simulink model "model_compatible"  (Simulink 7.5)
(part 5 of 5)

  Boundary___Perseus_1_CN_92348290_275000_CN_92343043_275000/RConn2 -- T_92343043_275000_Boundary_Substation/LConn2 -- _CN_92343043_275000_CN_191269219_275000/LConn2
  Boundary___Perseus_1_CN_92348290_275000_CN_92343043_275000/RConn3 -- T_92343043_275000_Boundary_Substation/LConn3 -- _CN_92343043_275000_CN_191269219_275000/LConn3 -- bus101/LConn1
  T_217505021__/LConn1 -- _CN_92348290_275000_CN_217505021_275000/RConn1
  T_217505021__/LConn2 -- _CN_92348290_275000_CN_217505021_275000/RConn2
  _CN_92348290_275000_CN_217505021_275000/RConn3 -- T_217505021__/LConn3 -- bus102/LConn1
  _CN_92343043_275000_CN_191269219_275000/RConn1 -- T_191269219_275000_/LConn1 -- _CN_200757306_275000_CN_191269219_275000/LConn1
  _CN_92343043_275000_CN_191269219_275000/RConn2 -- T_191269219_275000_/LConn2 -- _CN_200757306_275000_CN_191269219_275000/LConn2
  _CN_92343043_275000_CN_191269219_275000/RConn3 -- T_191269219_275000_/LConn3 -- _CN_200757306_275000_CN_191269219_275000/LConn3 -- bus103/LConn1
  T_230551819__/RConn1 -- _CN_230551819_275000_CN_182253896_275000/LConn1
  T_230551819__/RConn2 -- _CN_230551819_275000_CN_182253896_275000/LConn2
  _CN_230551819_275000_CN_182253896_275000/LConn3 -- T_230551819__/RConn3 -- bus104/LConn1
  _CN_230551819_275000_CN_182253896_275000/RConn1 -- T_182253896__/LConn1 -- _CN_182262936_275000_CN_182253896_275000/RConn1
  _CN_230551819_275000_CN_182253896_275000/RConn2 -- T_182253896__/LConn2 -- _CN_182262936_275000_CN_182253896_275000/RConn2
  _CN_230551819_275000_CN_182253896_275000/RConn3 -- T_182253896__/LConn3 -- _CN_182262936_275000_CN_182253896_275000/RConn3 -- bus105/LConn1
  _CN_184191239_275000_CN_107391770_275000/LConn1 -- T_184191239_275000_Illovo_Substation/LConn1 -- _CN_184191239_275000_CN_176259936_275000/LConn1
  _CN_184191239_275000_CN_107391770_275000/LConn2 -- T_184191239_275000_Illovo_Substation/LConn2 -- _CN_184191239_275000_CN_176259936_275000/LConn2
  _CN_184191239_275000_CN_107391770_275000/LConn3 -- T_184191239_275000_Illovo_Substation/LConn3 -- _CN_184191239_275000_CN_176259936_275000/LConn3 -- bus106/LConn1
  _CN_184191239_275000_CN_107391770_275000/RConn1 -- T_107391770_400000;275000_/RConn1 -- _CN_107391770_275000_CN_184187955_275000/LConn1 -- L_107391770/LConn1
  _CN_184191239_275000_CN_107391770_275000/RConn2 -- T_107391770_400000;275000_/RConn2 -- _CN_107391770_275000_CN_184187955_275000/LConn2 -- L_107391770/LConn2
  _CN_184191239_275000_CN_107391770_275000/RConn3 -- T_107391770_400000;275000_/RConn3 -- _CN_107391770_275000_CN_184187955_275000/LConn3 -- L_107391770/LConn3 -- bus107/LConn1
  _CN_184191239_275000_CN_176259936_275000/RConn1 -- T_176259936_275000_Georgedale_Substation/LConn1 -- _CN_184187955_275000_CN_176259936_275000/LConn1 -- _CN_181284056_275000_CN_176259936_275000/LConn1 -- _CN_127585817_275000_CN_176259936_275000/LConn1
  _CN_184191239_275000_CN_176259936_275000/RConn2 -- T_176259936_275000_Georgedale_Substation/LConn2 -- _CN_184187955_275000_CN_176259936_275000/LConn2 -- _CN_181284056_275000_CN_176259936_275000/LConn2 -- _CN_127585817_275000_CN_176259936_275000/LConn2
  _CN_184191239_275000_CN_176259936_275000/RConn3 -- T_176259936_275000_Georgedale_Substation/LConn3 -- _CN_184187955_275000_CN_176259936_275000/LConn3 -- _CN_181284056_275000_CN_176259936_275000/LConn3 -- bus108/LConn1 -- _CN_127585817_275000_CN_176259936_275000/LConn3
  T_184336448__/LConn1 -- _CN_184336448_275000_CN_87404898_275000/RConn1
  T_184336448__/LConn2 -- _CN_184336448_275000_CN_87404898_275000/RConn2
  _CN_184336448_275000_CN_87404898_275000/RConn3 -- T_184336448__/LConn3 -- bus109/LConn1
  T_84274092_380000;132000_/LConn1 -- _CN_84274092_275000_CN_83525879_275000/LConn1
  T_84274092_380000;132000_/LConn2 -- _CN_84274092_275000_CN_83525879_275000/LConn2
  _CN_84274092_275000_CN_83525879_275000/LConn3 -- T_84274092_380000;132000_/LConn3 -- bus110/LConn1
  _CN_84274092_275000_CN_83525879_275000/RConn1 -- T_83525879_400000;275000_Apollo_Substation/RConn1 -- _CN_28088740_275000_CN_83525879_275000/LConn1 -- _CN_83951788_275000_CN_83525879_275000/LConn1 -- _CN_83525876_275000_CN_83525879_275000/LConn1 -- L_83525879/LConn1
  _CN_84274092_275000_CN_83525879_275000/RConn2 -- T_83525879_400000;275000_Apollo_Substation/RConn2 -- _CN_28088740_275000_CN_83525879_275000/LConn2 -- _CN_83951788_275000_CN_83525879_275000/LConn2 -- _CN_83525876_275000_CN_83525879_275000/LConn2 -- L_83525879/LConn2
  _CN_84274092_275000_CN_83525879_275000/RConn3 -- T_83525879_400000;275000_Apollo_Substation/RConn3 -- _CN_28088740_275000_CN_83525879_275000/LConn3 -- _CN_83951788_275000_CN_83525879_275000/LConn3 -- _CN_83525876_275000_CN_83525879_275000/LConn3 -- L_83525879/LConn3 -- bus111/LConn1
  _CN_215459082_275000_CN_149126524_275000/LConn1 -- T_215459082_275000_Rigi_Substation/LConn1 -- _CN_215459082_275000_CN_98231341_275000/LConn1
  _CN_215459082_275000_CN_149126524_275000/LConn2 -- T_215459082_275000_Rigi_Substation/LConn2 -- _CN_215459082_275000_CN_98231341_275000/LConn2
  _CN_215459082_275000_CN_149126524_275000/LConn3 -- T_215459082_275000_Rigi_Substation/LConn3 -- _CN_215459082_275000_CN_98231341_275000/LConn3 -- bus112/LConn1
  _CN_215459082_275000_CN_149126524_275000/RConn1 -- T_149126524_275000_/LConn1 -- _CN_178252032_275000_CN_149126524_275000/LConn1 -- _CN_105811523_275000_CN_149126524_275000/LConn1
  _CN_215459082_275000_CN_149126524_275000/RConn2 -- T_149126524_275000_/LConn2 -- _CN_178252032_275000_CN_149126524_275000/LConn2 -- _CN_105811523_275000_CN_149126524_275000/LConn2
  _CN_215459082_275000_CN_149126524_275000/RConn3 -- T_149126524_275000_/LConn3 -- _CN_178252032_275000_CN_149126524_275000/LConn3 -- bus113/LConn1 -- _CN_105811523_275000_CN_149126524_275000/LConn3
  _CN_215459082_275000_CN_98231341_275000/RConn1 -- T_98231341_275000_/LConn1 -- _CN_98231341_275000_CN_214437948_275000/LConn1 -- _CN_98231341_275000_CN_136695854_275000/LConn1 -- _CN_98231341_275000_CN_105811523_275000/LConn1 -- _CN_98231341_275000_CN_81817181_275000/LConn1 -- _CN_98231341_275000_CN_189739076_275000/LConn1
  _CN_215459082_275000_CN_98231341_275000/RConn2 -- T_98231341_275000_/LConn2 -- _CN_98231341_275000_CN_214437948_275000/LConn2 -- _CN_98231341_275000_CN_136695854_275000/LConn2 -- _CN_98231341_275000_CN_105811523_275000/LConn2 -- _CN_98231341_275000_CN_81817181_275000/LConn2 -- _CN_98231341_275000_CN_189739076_275000/LConn2
  _CN_215459082_275000_CN_98231341_275000/RConn3 -- T_98231341_275000_/LConn3 -- _CN_98231341_275000_CN_214437948_275000/LConn3 -- _CN_98231341_275000_CN_136695854_275000/LConn3 -- _CN_98231341_275000_CN_105811523_275000/LConn3 -- _CN_98231341_275000_CN_81817181_275000/LConn3 -- _CN_98231341_275000_CN_189739076_275000/LConn3 -- bus114/LConn1
  _CN_183907671_275000_CN_181284049_275000/LConn1 -- T_183907671_275000;132000_Avon_Substation/LConn1 -- _CN_183907671_275000_CN_183907662_275000/LConn1
  _CN_183907671_275000_CN_181284049_275000/LConn2 -- T_183907671_275000;132000_Avon_Substation/LConn2 -- _CN_183907671_275000_CN_183907662_275000/LConn2
  _CN_183907671_275000_CN_181284049_275000/LConn3 -- T_183907671_275000;132000_Avon_Substation/LConn3 -- _CN_183907671_275000_CN_183907662_275000/LConn3 -- bus115/LConn1
  T_181284049__/RConn1 -- _CN_183907671_275000_CN_181284049_275000/RConn1
  T_181284049__/RConn2 -- _CN_183907671_275000_CN_181284049_275000/RConn2
  _CN_183907671_275000_CN_181284049_275000/RConn3 -- T_181284049__/RConn3 -- bus116/LConn1
  T_183907662_275000;132000_Ottawa_Substation/LConn1 -- _CN_183907671_275000_CN_183907662_275000/RConn1
  T_183907662_275000;132000_Ottawa_Substation/LConn2 -- _CN_183907671_275000_CN_183907662_275000/RConn2
  _CN_183907671_275000_CN_183907662_275000/RConn3 -- T_183907662_275000;132000_Ottawa_Substation/LConn3 -- bus117/LConn1
  T_184602696__/LConn1 -- _CN_184602696_275000_CN_184552955_275000/LConn1
  T_184602696__/LConn2 -- _CN_184602696_275000_CN_184552955_275000/LConn2
  _CN_184602696_275000_CN_184552955_275000/LConn3 -- T_184602696__/LConn3 -- bus118/LConn1
  _CN_184602696_275000_CN_184552955_275000/RConn1 -- T_184552955__/RConn1 -- _CN_258020275_275000_CN_184552955_275000/LConn1 -- _CN_184552955_275000_CN_208749745_275000/LConn1 -- L_184552955/LConn1
  _CN_184602696_275000_CN_184552955_275000/RConn2 -- T_184552955__/RConn2 -- _CN_258020275_275000_CN_184552955_275000/LConn2 -- _CN_184552955_275000_CN_208749745_275000/LConn2 -- L_184552955/LConn2
  _CN_184602696_275000_CN_184552955_275000/RConn3 -- T_184552955__/RConn3 -- _CN_258020275_275000_CN_184552955_275000/LConn3 -- _CN_184552955_275000_CN_208749745_275000/LConn3 -- L_184552955/LConn3 -- bus119/LConn1
  _CN_75136015_275000_CN_32509808_275000/LConn1 -- T_75136015_400000;275000_Minerva_Substation/RConn1 -- _CN_75136015_275000_CN_187432497_275000/LConn1 -- L_75136015/LConn1 -- _CN_75136015_275000_CN_178950118_275000/LConn1 -- _CN_75136015_275000_CN_84197405_275000/LConn1
  _CN_75136015_275000_CN_32509808_275000/LConn2 -- T_75136015_400000;275000_Minerva_Substation/RConn2 -- _CN_75136015_275000_CN_187432497_275000/LConn2 -- L_75136015/LConn2 -- _CN_75136015_275000_CN_178950118_275000/LConn2 -- _CN_75136015_275000_CN_84197405_275000/LConn2
  _CN_75136015_275000_CN_32509808_275000/LConn3 -- T_75136015_400000;275000_Minerva_Substation/RConn3 -- _CN_75136015_275000_CN_187432497_275000/LConn3 -- L_75136015/LConn3 -- bus120/LConn1 -- _CN_75136015_275000_CN_178950118_275000/LConn3 -- _CN_75136015_275000_CN_84197405_275000/LConn3
  _CN_75136015_275000_CN_32509808_275000/RConn1 -- T_32509808__Lepini_Substation/LConn1 -- _CN_178950118_275000_CN_32509808_275000/LConn1
  _CN_75136015_275000_CN_32509808_275000/RConn2 -- T_32509808__Lepini_Substation/LConn2 -- _CN_178950118_275000_CN_32509808_275000/LConn2
  _CN_75136015_275000_CN_32509808_275000/RConn3 -- T_32509808__Lepini_Substation/LConn3 -- _CN_178950118_275000_CN_32509808_275000/LConn3 -- bus121/LConn1
  _CN_75136015_275000_CN_178950118_275000/RConn1 -- T_178950118_275000_Craighall_Substation/LConn1 -- _CN_178950118_275000_CN_32509808_275000/RConn1
  _CN_75136015_275000_CN_178950118_275000/RConn2 -- T_178950118_275000_Craighall_Substation/LConn2 -- _CN_178950118_275000_CN_32509808_275000/RConn2
  _CN_75136015_275000_CN_178950118_275000/RConn3 -- T_178950118_275000_Craighall_Substation/LConn3 -- _CN_178950118_275000_CN_32509808_275000/RConn3 -- bus122/LConn1
  T_84197405_380000;132000_/LConn1 -- _CN_75136015_275000_CN_84197405_275000/RConn1
  T_84197405_380000;132000_/LConn2 -- _CN_75136015_275000_CN_84197405_275000/RConn2
  _CN_75136015_275000_CN_84197405_275000/RConn3 -- T_84197405_380000;132000_/LConn3 -- bus123/LConn1
  T_187432497__/LConn1 -- _CN_75136015_275000_CN_187432497_275000/RConn1
  T_187432497__/LConn2 -- _CN_75136015_275000_CN_187432497_275000/RConn2
  _CN_75136015_275000_CN_187432497_275000/RConn3 -- T_187432497__/LConn3 -- bus124/LConn1
  _CN_156418705_275000_CN_136019706_275000/RConn1 -- T_136019706__/LConn1 -- _CN_135726365_275000_CN_136019706_275000/LConn1
  _CN_156418705_275000_CN_136019706_275000/RConn2 -- T_136019706__/LConn2 -- _CN_135726365_275000_CN_136019706_275000/LConn2
  _CN_156418705_275000_CN_136019706_275000/RConn3 -- T_136019706__/LConn3 -- _CN_135726365_275000_CN_136019706_275000/LConn3 -- bus125/LConn1
  T_247956792__/LConn1 -- _CN_247956792_275000_CN_183764510_275000/LConn1
  T_247956792__/LConn2 -- _CN_247956792_275000_CN_183764510_275000/LConn2
  _CN_247956792_275000_CN_183764510_275000/LConn3 -- T_247956792__/LConn3 -- bus126/LConn1
  T_183764510__/LConn1 -- _CN_247956792_275000_CN_183764510_275000/RConn1
  T_183764510__/LConn2 -- _CN_247956792_275000_CN_183764510_275000/RConn2
  _CN_247956792_275000_CN_183764510_275000/RConn3 -- T_183764510__/LConn3 -- bus127/LConn1
  _CN_178987907_275000_CN_418832508_275000/RConn1 -- G_418832508_Arnot_Power_Station/RConn1 -- _CN_156418705_400000_CN_418832508_275000/LConn1 -- _CN_170672051_400000_CN_418832508_275000/LConn1 -- _CN_209976655_400000_CN_418832508_275000/LConn1 -- _CN_220129604_400000_CN_418832508_275000/LConn1
  _CN_178987907_275000_CN_418832508_275000/RConn2 -- G_418832508_Arnot_Power_Station/RConn2 -- _CN_156418705_400000_CN_418832508_275000/LConn2 -- _CN_170672051_400000_CN_418832508_275000/LConn2 -- _CN_209976655_400000_CN_418832508_275000/LConn2 -- _CN_220129604_400000_CN_418832508_275000/LConn2
  _CN_178987907_275000_CN_418832508_275000/RConn3 -- G_418832508_Arnot_Power_Station/RConn3 -- _CN_156418705_400000_CN_418832508_275000/LConn3 -- _CN_170672051_400000_CN_418832508_275000/LConn3 -- _CN_209976655_400000_CN_418832508_275000/LConn3 -- _CN_220129604_400000_CN_418832508_275000/LConn3 -- bus128/LConn1
  T_363326105__/LConn1 -- _CN_363326105_275000_CN_179856840_275000/LConn1
  T_363326105__/LConn2 -- _CN_363326105_275000_CN_179856840_275000/LConn2
  _CN_363326105_275000_CN_179856840_275000/LConn3 -- T_363326105__/LConn3 -- bus129/LConn1
  T_179856840_275000_Komatipoort_Substation/LConn1 -- _CN_363326105_275000_CN_179856840_275000/RConn1
  T_179856840_275000_Komatipoort_Substation/LConn2 -- _CN_363326105_275000_CN_179856840_275000/RConn2
  _CN_363326105_275000_CN_179856840_275000/RConn3 -- T_179856840_275000_Komatipoort_Substation/LConn3 -- bus130/LConn1
  _CN_127585817_275000_CN_176259936_275000/RConn1 -- T_127585817__/RConn1 -- _CN_127585817_275000_CN_148830396_275000/LConn1 -- L_127585817/LConn1
  _CN_127585817_275000_CN_176259936_275000/RConn2 -- T_127585817__/RConn2 -- _CN_127585817_275000_CN_148830396_275000/LConn2 -- L_127585817/LConn2
  _CN_127585817_275000_CN_176259936_275000/RConn3 -- T_127585817__/RConn3 -- _CN_127585817_275000_CN_148830396_275000/LConn3 -- L_127585817/LConn3 -- bus131/LConn1
  _CN_127585817_275000_CN_148830396_275000/RConn1 -- T_148830396__/LConn1 -- _CN_104071861_275000_CN_148830396_275000/LConn1
  _CN_127585817_275000_CN_148830396_275000/RConn2 -- T_148830396__/LConn2 -- _CN_104071861_275000_CN_148830396_275000/LConn2
  _CN_127585817_275000_CN_148830396_275000/RConn3 -- T_148830396__/LConn3 -- _CN_104071861_275000_CN_148830396_275000/LConn3 -- bus132/LConn1
  _CN_84391364_275000_CN_136695854_275000/LConn1 -- T_84391364_275000_Nevis_Substation/LConn1 -- _CN_84391364_275000_CN_418842091_275000/LConn1 -- _CN_84391364_275000_CN_136695855_275000/LConn1
  _CN_84391364_275000_CN_136695854_275000/LConn2 -- T_84391364_275000_Nevis_Substation/LConn2 -- _CN_84391364_275000_CN_418842091_275000/LConn2 -- _CN_84391364_275000_CN_136695855_275000/LConn2
  _CN_84391364_275000_CN_136695854_275000/LConn3 -- T_84391364_275000_Nevis_Substation/LConn3 -- _CN_84391364_275000_CN_418842091_275000/LConn3 -- bus133/LConn1 -- _CN_84391364_275000_CN_136695855_275000/LConn3
  _CN_84391364_275000_CN_136695854_275000/RConn1 -- T_136695854__/LConn1 -- _CN_98231341_275000_CN_136695854_275000/RConn1
  _CN_84391364_275000_CN_136695854_275000/RConn2 -- T_136695854__/LConn2 -- _CN_98231341_275000_CN_136695854_275000/RConn2
  _CN_84391364_275000_CN_136695854_275000/RConn3 -- T_136695854__/LConn3 -- _CN_98231341_275000_CN_136695854_275000/RConn3 -- bus134/LConn1
  T_136695855__/LConn1 -- _CN_84391364_275000_CN_136695855_275000/RConn1
  T_136695855__/LConn2 -- _CN_84391364_275000_CN_136695855_275000/RConn2
  _CN_84391364_275000_CN_136695855_275000/RConn3 -- T_136695855__/LConn3 -- bus135/LConn1
  _CN_84391364_275000_CN_418842091_275000/RConn1 -- G_418842091_Matla_Power_Station/RConn1 -- _CN_185481654_275000_CN_418842091_275000/LConn1 -- _CN_83950316_275000_CN_418842091_275000/LConn1
  _CN_84391364_275000_CN_418842091_275000/RConn2 -- G_418842091_Matla_Power_Station/RConn2 -- _CN_185481654_275000_CN_418842091_275000/LConn2 -- _CN_83950316_275000_CN_418842091_275000/LConn2
  _CN_84391364_275000_CN_418842091_275000/RConn3 -- G_418842091_Matla_Power_Station/RConn3 -- _CN_185481654_275000_CN_418842091_275000/LConn3 -- _CN_83950316_275000_CN_418842091_275000/LConn3 -- bus136/LConn1
  _CN_107391770_275000_CN_184187955_275000/RConn1 -- T_184187955_275000_Klaarwater_Substation/LConn1 -- _CN_197060002_275000_CN_184187955_275000/LConn1 -- _CN_184187955_275000_CN_176259936_275000/RConn1
  _CN_107391770_275000_CN_184187955_275000/RConn2 -- T_184187955_275000_Klaarwater_Substation/LConn2 -- _CN_197060002_275000_CN_184187955_275000/LConn2 -- _CN_184187955_275000_CN_176259936_275000/RConn2
  _CN_107391770_275000_CN_184187955_275000/RConn3 -- T_184187955_275000_Klaarwater_Substation/LConn3 -- _CN_197060002_275000_CN_184187955_275000/LConn3 -- _CN_184187955_275000_CN_176259936_275000/RConn3 -- bus137/LConn1
  T_178240540__/LConn1 -- _CN_178240540_275000_CN_83188568_275000/LConn1
  T_178240540__/LConn2 -- _CN_178240540_275000_CN_83188568_275000/LConn2
  _CN_178240540_275000_CN_83188568_275000/LConn3 -- T_178240540__/LConn3 -- bus138/LConn1
  _CN_178240540_275000_CN_83188568_275000/RConn1 -- T_83188568_275000;132000_Taunus_Substation/LConn1 -- _CN_178240552_275000_CN_83188568_275000/LConn1 -- _CN_83888980_275000_CN_83188568_275000/LConn1 -- _CN_82014905_275000_CN_83188568_275000/LConn1
  _CN_178240540_275000_CN_83188568_275000/RConn2 -- T_83188568_275000;132000_Taunus_Substation/LConn2 -- _CN_178240552_275000_CN_83188568_275000/LConn2 -- _CN_83888980_275000_CN_83188568_275000/LConn2 -- _CN_82014905_275000_CN_83188568_275000/LConn2
  _CN_178240540_275000_CN_83188568_275000/RConn3 -- T_83188568_275000;132000_Taunus_Substation/LConn3 -- _CN_178240552_275000_CN_83188568_275000/LConn3 -- _CN_83888980_275000_CN_83188568_275000/LConn3 -- _CN_82014905_275000_CN_83188568_275000/LConn3 -- bus139/LConn1
  T_100421919__/LConn1 -- _CN_100421919_275000_CN_200757306_275000/LConn1
  T_100421919__/LConn2 -- _CN_100421919_275000_CN_200757306_275000/LConn2
  _CN_100421919_275000_CN_200757306_275000/LConn3 -- T_100421919__/LConn3 -- bus140/LConn1
  _CN_100421919_275000_CN_200757306_275000/RConn1 -- T_200757306__/LConn1 -- _CN_200757306_275000_CN_191269219_275000/RConn1
  _CN_100421919_275000_CN_200757306_275000/RConn2 -- T_200757306__/LConn2 -- _CN_200757306_275000_CN_191269219_275000/RConn2
  _CN_100421919_275000_CN_200757306_275000/RConn3 -- T_200757306__/LConn3 -- _CN_200757306_275000_CN_191269219_275000/RConn3 -- bus141/LConn1
  _CN_131625968_275000_CN_120941257_275000/LConn1 -- T_131625968_132000_Nseleni_Substation/RConn1 -- L_131625968/LConn1
  _CN_131625968_275000_CN_120941257_275000/LConn2 -- T_131625968_132000_Nseleni_Substation/RConn2 -- L_131625968/LConn2
  _CN_131625968_275000_CN_120941257_275000/LConn3 -- T_131625968_132000_Nseleni_Substation/RConn3 -- L_131625968/LConn3 -- bus142/LConn1
  T_120941257_275000;132000_Impala_Substation/LConn1 -- _CN_131625968_275000_CN_120941257_275000/RConn1
  T_120941257_275000;132000_Impala_Substation/LConn2 -- _CN_131625968_275000_CN_120941257_275000/RConn2
  _CN_131625968_275000_CN_120941257_275000/RConn3 -- T_120941257_275000;132000_Impala_Substation/LConn3 -- bus143/LConn1
  T_197060002__/LConn1 -- _CN_197060002_275000_CN_184187955_275000/RConn1
  T_197060002__/LConn2 -- _CN_197060002_275000_CN_184187955_275000/RConn2
  _CN_197060002_275000_CN_184187955_275000/RConn3 -- T_197060002__/LConn3 -- bus144/LConn1
  _CN_220129604_275000_CN_101150274_275000/LConn1 -- T_220129604_400000_Arnot_Power_Station/RConn1 -- _CN_220129604_275000_CN_138280477_275000/LConn1 -- L_220129604/LConn1
  _CN_220129604_275000_CN_101150274_275000/LConn2 -- T_220129604_400000_Arnot_Power_Station/RConn2 -- _CN_220129604_275000_CN_138280477_275000/LConn2 -- L_220129604/LConn2
  _CN_220129604_275000_CN_101150274_275000/LConn3 -- T_220129604_400000_Arnot_Power_Station/RConn3 -- _CN_220129604_275000_CN_138280477_275000/LConn3 -- L_220129604/LConn3 -- bus145/LConn1
  _CN_220129604_275000_CN_101150274_275000/RConn1 -- T_101150274__/LConn1 -- _CN_93158442_275000_CN_101150274_275000/LConn1
  _CN_220129604_275000_CN_101150274_275000/RConn2 -- T_101150274__/LConn2 -- _CN_93158442_275000_CN_101150274_275000/LConn2
  _CN_220129604_275000_CN_101150274_275000/RConn3 -- T_101150274__/LConn3 -- _CN_93158442_275000_CN_101150274_275000/LConn3 -- bus146/LConn1
  T_138280477__/LConn1 -- _CN_220129604_275000_CN_138280477_275000/RConn1
  T_138280477__/LConn2 -- _CN_220129604_275000_CN_138280477_275000/RConn2
  _CN_220129604_275000_CN_138280477_275000/RConn3 -- T_138280477__/LConn3 -- bus147/LConn1
  _CN_28088740_275000_CN_83525879_275000/RConn1 -- T_28088740_275000_Croydon_Substation/LConn1 -- _CN_28088740_275000_CN_42209860_275000/LConn1
  _CN_28088740_275000_CN_83525879_275000/RConn2 -- T_28088740_275000_Croydon_Substation/LConn2 -- _CN_28088740_275000_CN_42209860_275000/LConn2
  _CN_28088740_275000_CN_83525879_275000/RConn3 -- T_28088740_275000_Croydon_Substation/LConn3 -- _CN_28088740_275000_CN_42209860_275000/LConn3 -- bus148/LConn1
  _CN_28088740_275000_CN_42209860_275000/RConn1 -- T_42209860_275000_Jupiter_Substation/LConn1 -- _CN_42209860_275000_CN_42209493_275000/LConn1 -- _CN_42209860_275000_CN_178944143_275000/LConn1
  _CN_28088740_275000_CN_42209860_275000/RConn2 -- T_42209860_275000_Jupiter_Substation/LConn2 -- _CN_42209860_275000_CN_42209493_275000/LConn2 -- _CN_42209860_275000_CN_178944143_275000/LConn2
  _CN_28088740_275000_CN_42209860_275000/RConn3 -- T_42209860_275000_Jupiter_Substation/LConn3 -- _CN_42209860_275000_CN_42209493_275000/LConn3 -- _CN_42209860_275000_CN_178944143_275000/LConn3 -- bus149/LConn1
  _CN_178240552_275000_CN_105811523_275000/LConn1 -- T_178240552__/LConn1 -- _CN_178240552_275000_CN_83945972_275000/LConn1 -- _CN_178240552_275000_CN_83188568_275000/RConn1
  _CN_178240552_275000_CN_105811523_275000/LConn2 -- T_178240552__/LConn2 -- _CN_178240552_275000_CN_83945972_275000/LConn2 -- _CN_178240552_275000_CN_83188568_275000/RConn2
  _CN_178240552_275000_CN_105811523_275000/LConn3 -- T_178240552__/LConn3 -- _CN_178240552_275000_CN_83945972_275000/LConn3 -- _CN_178240552_275000_CN_83188568_275000/RConn3 -- bus150/LConn1
  _CN_178240552_275000_CN_105811523_275000/RConn1 -- T_105811523_400000;275000_Glockner_Substation/RConn1 -- _CN_98231341_275000_CN_105811523_275000/RConn1 -- _CN_105811509_275000_CN_105811523_275000/LConn1 -- _CN_105811523_275000_CN_178248302_275000/LConn1 -- _CN_105811523_275000_CN_149126524_275000/RConn1 -- L_105811523/LConn1
  _CN_178240552_275000_CN_105811523_275000/RConn2 -- T_105811523_400000;275000_Glockner_Substation/RConn2 -- _CN_98231341_275000_CN_105811523_275000/RConn2 -- _CN_105811509_275000_CN_105811523_275000/LConn2 -- _CN_105811523_275000_CN_178248302_275000/LConn2 -- _CN_105811523_275000_CN_149126524_275000/RConn2 -- L_105811523/LConn2
  _CN_178240552_275000_CN_105811523_275000/RConn3 -- T_105811523_400000;275000_Glockner_Substation/RConn3 -- _CN_98231341_275000_CN_105811523_275000/RConn3 -- _CN_105811509_275000_CN_105811523_275000/LConn3 -- _CN_105811523_275000_CN_178248302_275000/LConn3 -- _CN_105811523_275000_CN_149126524_275000/RConn3 -- L_105811523/LConn3 -- bus151/LConn1
  _CN_178240552_275000_CN_83945972_275000/RConn1 -- T_83945972__/LConn1 -- _CN_83888980_275000_CN_83945972_275000/LConn1
  _CN_178240552_275000_CN_83945972_275000/RConn2 -- T_83945972__/LConn2 -- _CN_83888980_275000_CN_83945972_275000/LConn2
  _CN_178240552_275000_CN_83945972_275000/RConn3 -- T_83945972__/LConn3 -- _CN_83888980_275000_CN_83945972_275000/LConn3 -- bus152/LConn1
  T_93158442_275000_Marathon_Substation/LConn1 -- _CN_93158442_275000_CN_101150274_275000/RConn1
  T_93158442_275000_Marathon_Substation/LConn2 -- _CN_93158442_275000_CN_101150274_275000/RConn2
  _CN_93158442_275000_CN_101150274_275000/RConn3 -- T_93158442_275000_Marathon_Substation/LConn3 -- bus153/LConn1
  _CN_83951788_275000_CN_83525879_275000/RConn1 -- T_83951788_275000_Esselen_Substation/LConn1 -- _CN_83951788_275000_CN_178983951_275000/LConn1
  _CN_83951788_275000_CN_83525879_275000/RConn2 -- T_83951788_275000_Esselen_Substation/LConn2 -- _CN_83951788_275000_CN_178983951_275000/LConn2
  _CN_83951788_275000_CN_83525879_275000/RConn3 -- T_83951788_275000_Esselen_Substation/LConn3 -- _CN_83951788_275000_CN_178983951_275000/LConn3 -- bus154/LConn1
  _CN_83951788_275000_CN_178983951_275000/RConn1 -- T_178983951__/LConn1 -- _CN_258020275_275000_CN_178983951_275000/LConn1
  _CN_83951788_275000_CN_178983951_275000/RConn2 -- T_178983951__/LConn2 -- _CN_258020275_275000_CN_178983951_275000/LConn2
  _CN_83951788_275000_CN_178983951_275000/RConn3 -- T_178983951__/LConn3 -- _CN_258020275_275000_CN_178983951_275000/LConn3 -- bus155/LConn1
  _CN_98231341_275000_CN_214437948_275000/RConn1 -- T_214437948_275000_Brenner_Substation/LConn1 -- _CN_214437948_275000_CN_81817181_275000/LConn1
  _CN_98231341_275000_CN_214437948_275000/RConn2 -- T_214437948_275000_Brenner_Substation/LConn2 -- _CN_214437948_275000_CN_81817181_275000/LConn2
  _CN_98231341_275000_CN_214437948_275000/RConn3 -- T_214437948_275000_Brenner_Substation/LConn3 -- _CN_214437948_275000_CN_81817181_275000/LConn3 -- bus156/LConn1
  _CN_98231341_275000_CN_81817181_275000/RConn1 -- T_81817181_275000_Eiger_Substation/LConn1 -- _CN_82014905_275000_CN_81817181_275000/LConn1 -- _CN_178944143_275000_CN_81817181_275000/LConn1 -- _CN_214437948_275000_CN_81817181_275000/RConn1 -- _CN_42209493_275000_CN_81817181_275000/LConn1
  _CN_98231341_275000_CN_81817181_275000/RConn2 -- T_81817181_275000_Eiger_Substation/LConn2 -- _CN_82014905_275000_CN_81817181_275000/LConn2 -- _CN_178944143_275000_CN_81817181_275000/LConn2 -- _CN_214437948_275000_CN_81817181_275000/RConn2 -- _CN_42209493_275000_CN_81817181_275000/LConn2
  _CN_98231341_275000_CN_81817181_275000/RConn3 -- T_81817181_275000_Eiger_Substation/LConn3 -- _CN_82014905_275000_CN_81817181_275000/LConn3 -- _CN_178944143_275000_CN_81817181_275000/LConn3 -- bus157/LConn1 -- _CN_214437948_275000_CN_81817181_275000/RConn3 -- _CN_42209493_275000_CN_81817181_275000/LConn3
  _CN_98231341_275000_CN_189739076_275000/RConn1 -- T_189739076_275000_Makalu_Substation/LConn1 -- _CN_189739076_275000_CN_178252032_275000/LConn1
  _CN_98231341_275000_CN_189739076_275000/RConn2 -- T_189739076_275000_Makalu_Substation/LConn2 -- _CN_189739076_275000_CN_178252032_275000/LConn2
  _CN_98231341_275000_CN_189739076_275000/RConn3 -- T_189739076_275000_Makalu_Substation/LConn3 -- _CN_189739076_275000_CN_178252032_275000/LConn3 -- bus158/LConn1
  T_135726365__/LConn1 -- _CN_135726365_275000_CN_136019706_275000/RConn1
  T_135726365__/LConn2 -- _CN_135726365_275000_CN_136019706_275000/RConn2
  _CN_135726365_275000_CN_136019706_275000/RConn3 -- T_135726365__/LConn3 -- bus159/LConn1
  T_104071861__/LConn1 -- _CN_104071861_275000_CN_148830396_275000/RConn1
  T_104071861__/LConn2 -- _CN_104071861_275000_CN_148830396_275000/RConn2
  _CN_104071861_275000_CN_148830396_275000/RConn3 -- T_104071861__/LConn3 -- bus160/LConn1
  _CN_185481654_275000_CN_185341298_275000/LConn1 -- T_185481654__/LConn1 -- _CN_185481654_275000_CN_209979772_275000/LConn1 -- _CN_185481654_275000_CN_418842091_275000/RConn1
  _CN_185481654_275000_CN_185341298_275000/LConn2 -- T_185481654__/LConn2 -- _CN_185481654_275000_CN_209979772_275000/LConn2 -- _CN_185481654_275000_CN_418842091_275000/RConn2
  _CN_185481654_275000_CN_185341298_275000/LConn3 -- T_185481654__/LConn3 -- _CN_185481654_275000_CN_209979772_275000/LConn3 -- _CN_185481654_275000_CN_418842091_275000/RConn3 -- bus161/LConn1
  G_185341298_/RConn1 -- _CN_185481654_275000_CN_185341298_275000/RConn1
  G_185341298_/RConn2 -- _CN_185481654_275000_CN_185341298_275000/RConn2
  _CN_185481654_275000_CN_185341298_275000/RConn3 -- G_185341298_/RConn3 -- bus162/LConn1
  T_209979772__/LConn1 -- _CN_185481654_275000_CN_209979772_275000/RConn1
  T_209979772__/LConn2 -- _CN_185481654_275000_CN_209979772_275000/RConn2
  _CN_185481654_275000_CN_209979772_275000/RConn3 -- T_209979772__/LConn3 -- bus163/LConn1
  T_181284056_275000_/LConn1 -- _CN_181284056_275000_CN_176259936_275000/RConn1
  T_181284056_275000_/LConn2 -- _CN_181284056_275000_CN_176259936_275000/RConn2
  _CN_181284056_275000_CN_176259936_275000/RConn3 -- T_181284056_275000_/LConn3 -- bus164/LConn1
  T_83525876__/LConn1 -- _CN_83525876_275000_CN_83525879_275000/RConn1
  T_83525876__/LConn2 -- _CN_83525876_275000_CN_83525879_275000/RConn2
  _CN_83525876_275000_CN_83525879_275000/RConn3 -- T_83525876__/LConn3 -- bus165/LConn1
  T_105811509_275000_Verdun_Substation/LConn1 -- _CN_105811509_275000_CN_105811523_275000/RConn1
  T_105811509_275000_Verdun_Substation/LConn2 -- _CN_105811509_275000_CN_105811523_275000/RConn2
  _CN_105811509_275000_CN_105811523_275000/RConn3 -- T_105811509_275000_Verdun_Substation/LConn3 -- bus166/LConn1
  T_178248302_275000_Kookfontein_Substation/LConn1 -- _CN_105811523_275000_CN_178248302_275000/RConn1
  T_178248302_275000_Kookfontein_Substation/LConn2 -- _CN_105811523_275000_CN_178248302_275000/RConn2
  _CN_105811523_275000_CN_178248302_275000/RConn3 -- T_178248302_275000_Kookfontein_Substation/LConn3 -- bus167/LConn1
  _CN_42209860_275000_CN_42209493_275000/RConn1 -- T_42209493_275000;132000_Prospec_Substation/LConn1 -- _CN_42209493_275000_CN_81817181_275000/RConn1
  _CN_42209860_275000_CN_42209493_275000/RConn2 -- T_42209493_275000;132000_Prospec_Substation/LConn2 -- _CN_42209493_275000_CN_81817181_275000/RConn2
  _CN_42209860_275000_CN_42209493_275000/RConn3 -- T_42209493_275000;132000_Prospec_Substation/LConn3 -- _CN_42209493_275000_CN_81817181_275000/RConn3 -- bus168/LConn1
  _CN_42209860_275000_CN_178944143_275000/RConn1 -- T_178944143_275000_Fordsburg_Substation/LConn1 -- _CN_178944143_275000_CN_81817181_275000/RConn1
  _CN_42209860_275000_CN_178944143_275000/RConn2 -- T_178944143_275000_Fordsburg_Substation/LConn2 -- _CN_178944143_275000_CN_81817181_275000/RConn2
  _CN_42209860_275000_CN_178944143_275000/RConn3 -- T_178944143_275000_Fordsburg_Substation/LConn3 -- _CN_178944143_275000_CN_81817181_275000/RConn3 -- bus169/LConn1
  _CN_189739076_275000_CN_178252032_275000/RConn1 -- T_178252032_275000_Scafell_Substation/LConn1 -- _CN_178252032_275000_CN_149126524_275000/RConn1
  _CN_189739076_275000_CN_178252032_275000/RConn2 -- T_178252032_275000_Scafell_Substation/LConn2 -- _CN_178252032_275000_CN_149126524_275000/RConn2
  _CN_189739076_275000_CN_178252032_275000/RConn3 -- T_178252032_275000_Scafell_Substation/LConn3 -- _CN_178252032_275000_CN_149126524_275000/RConn3 -- bus170/LConn1
  _CN_83888980_275000_CN_83188568_275000/RConn1 -- T_83888980__/LConn1 -- _CN_83888980_275000_CN_83945972_275000/RConn1
  _CN_83888980_275000_CN_83188568_275000/RConn2 -- T_83888980__/LConn2 -- _CN_83888980_275000_CN_83945972_275000/RConn2
  _CN_83888980_275000_CN_83188568_275000/RConn3 -- T_83888980__/LConn3 -- _CN_83888980_275000_CN_83945972_275000/RConn3 -- bus171/LConn1
  _CN_258020275_275000_CN_178983951_275000/RConn1 -- T_258020275__/LConn1 -- _CN_258020275_275000_CN_184552955_275000/RConn1
  _CN_258020275_275000_CN_178983951_275000/RConn2 -- T_258020275__/LConn2 -- _CN_258020275_275000_CN_184552955_275000/RConn2
  _CN_258020275_275000_CN_178983951_275000/RConn3 -- T_258020275__/LConn3 -- _CN_258020275_275000_CN_184552955_275000/RConn3 -- bus172/LConn1
  _CN_82014905_275000_CN_81817181_275000/RConn1 -- T_82014905_275000_Etna_Substation/LConn1 -- _CN_82014905_275000_CN_83188568_275000/RConn1
  _CN_82014905_275000_CN_81817181_275000/RConn2 -- T_82014905_275000_Etna_Substation/LConn2 -- _CN_82014905_275000_CN_83188568_275000/RConn2
  _CN_82014905_275000_CN_81817181_275000/RConn3 -- T_82014905_275000_Etna_Substation/LConn3 -- _CN_82014905_275000_CN_83188568_275000/RConn3 -- bus173/LConn1
  T_208749745__/LConn1 -- _CN_184552955_275000_CN_208749745_275000/RConn1
  T_208749745__/LConn2 -- _CN_184552955_275000_CN_208749745_275000/RConn2
  _CN_184552955_275000_CN_208749745_275000/RConn3 -- T_208749745__/LConn3 -- bus174/LConn1
  T_83950316_275000_Benburg_Substation/LConn1 -- _CN_83950316_275000_CN_418842091_275000/RConn1
  T_83950316_275000_Benburg_Substation/LConn2 -- _CN_83950316_275000_CN_418842091_275000/RConn2
  _CN_83950316_275000_CN_418842091_275000/RConn3 -- T_83950316_275000_Benburg_Substation/LConn3 -- bus175/LConn1
  _CN_176940672_400000_CN_230551819_400000/LConn1 -- T_176940672__/LConn1 -- _CN_176940672_400000_CN_184581460_400000/LConn1
  _CN_176940672_400000_CN_230551819_400000/LConn2 -- T_176940672__/LConn2 -- _CN_176940672_400000_CN_184581460_400000/LConn2
  _CN_176940672_400000_CN_230551819_400000/LConn3 -- T_176940672__/LConn3 -- _CN_176940672_400000_CN_184581460_400000/LConn3 -- bus176/LConn1
  _CN_176940672_400000_CN_230551819_400000/RConn1 -- T_230551819__/LConn1 -- _CN_230551819_400000_CN_182408147_400000/LConn1
  _CN_176940672_400000_CN_230551819_400000/RConn2 -- T_230551819__/LConn2 -- _CN_230551819_400000_CN_182408147_400000/LConn2
  _CN_176940672_400000_CN_230551819_400000/RConn3 -- T_230551819__/LConn3 -- _CN_230551819_400000_CN_182408147_400000/LConn3 -- bus177/LConn1
  _CN_176940672_400000_CN_184581460_400000/RConn1 -- T_184581460__/LConn1 -- _CN_184581460_400000_CN_83525879_400000/LConn1
  _CN_176940672_400000_CN_184581460_400000/RConn2 -- T_184581460__/LConn2 -- _CN_184581460_400000_CN_83525879_400000/LConn2
  _CN_176940672_400000_CN_184581460_400000/RConn3 -- T_184581460__/LConn3 -- _CN_184581460_400000_CN_83525879_400000/LConn3 -- bus178/LConn1
  _CN_185497473_400000_CN_83525879_400000/LConn1 -- T_185497473__/LConn1 -- _CN_185497473_400000_CN_185171511_400000/LConn1 -- _CN_185497473_400000_CN_178968761_400000/LConn1 -- _CN_185497473_400000_CN_75136015_400000/LConn1
  _CN_185497473_400000_CN_83525879_400000/LConn2 -- T_185497473__/LConn2 -- _CN_185497473_400000_CN_185171511_400000/LConn2 -- _CN_185497473_400000_CN_178968761_400000/LConn2 -- _CN_185497473_400000_CN_75136015_400000/LConn2
  _CN_185497473_400000_CN_83525879_400000/LConn3 -- T_185497473__/LConn3 -- _CN_185497473_400000_CN_185171511_400000/LConn3 -- _CN_185497473_400000_CN_178968761_400000/LConn3 -- _CN_185497473_400000_CN_75136015_400000/LConn3 -- bus179/LConn1
  _CN_185497473_400000_CN_83525879_400000/RConn1 -- T_83525879_400000;275000_Apollo_Substation/LConn1 -- _CN_75136015_400000_CN_83525879_400000/LConn1 -- _CN_170672051_400000_CN_83525879_400000/LConn1 -- _CN_185171518_400000_CN_83525879_400000/LConn1 -- _CN_184581460_400000_CN_83525879_400000/RConn1
  _CN_185497473_400000_CN_83525879_400000/RConn2 -- T_83525879_400000;275000_Apollo_Substation/LConn2 -- _CN_75136015_400000_CN_83525879_400000/LConn2 -- _CN_170672051_400000_CN_83525879_400000/LConn2 -- _CN_185171518_400000_CN_83525879_400000/LConn2 -- _CN_184581460_400000_CN_83525879_400000/RConn2
  _CN_185497473_400000_CN_83525879_400000/RConn3 -- T_83525879_400000;275000_Apollo_Substation/LConn3 -- _CN_75136015_400000_CN_83525879_400000/LConn3 -- bus180/LConn1 -- _CN_170672051_400000_CN_83525879_400000/LConn3 -- _CN_185171518_400000_CN_83525879_400000/LConn3 -- _CN_184581460_400000_CN_83525879_400000/RConn3
  _CN_185497473_400000_CN_185171511_400000/RConn1 -- G_185171511_Duvha_Power_Station/RConn1 -- _CN_184560833_400000_CN_185171511_400000/LConn1 -- _CN_238322344_400000_CN_185171511_400000/LConn1 -- _CN_170672051_400000_CN_185171511_400000/LConn1 -- _CN_65600948_400000_CN_185171511_400000/LConn1 -- _CN_185171518_400000_CN_185171511_400000/LConn1
  _CN_185497473_400000_CN_185171511_400000/RConn2 -- G_185171511_Duvha_Power_Station/RConn2 -- _CN_184560833_400000_CN_185171511_400000/LConn2 -- _CN_238322344_400000_CN_185171511_400000/LConn2 -- _CN_170672051_400000_CN_185171511_400000/LConn2 -- _CN_65600948_400000_CN_185171511_400000/LConn2 -- _CN_185171518_400000_CN_185171511_400000/LConn2
  _CN_185497473_400000_CN_185171511_400000/RConn3 -- G_185171511_Duvha_Power_Station/RConn3 -- _CN_184560833_400000_CN_185171511_400000/LConn3 -- _CN_238322344_400000_CN_185171511_400000/LConn3 -- _CN_170672051_400000_CN_185171511_400000/LConn3 -- _CN_65600948_400000_CN_185171511_400000/LConn3 -- _CN_185171518_400000_CN_185171511_400000/LConn3 -- bus181/LConn1
  _CN_185497473_400000_CN_178968761_400000/RConn1 -- T_178968761_765000;400000_/RConn1 -- _CN_98231311_400000_CN_178968761_400000/LConn1 -- _CN_179140081_400000_CN_178968761_400000/LConn1 -- _CN_65600948_400000_CN_178968761_400000/LConn1 -- _CN_178968761_400000_CN_98218556_400000/LConn1 -- _CN_178968761_400000_CN_418832515_400000/LConn1 -- L_178968761/LConn1
  _CN_185497473_400000_CN_178968761_400000/RConn2 -- T_178968761_765000;400000_/RConn2 -- _CN_98231311_400000_CN_178968761_400000/LConn2 -- _CN_179140081_400000_CN_178968761_400000/LConn2 -- _CN_65600948_400000_CN_178968761_400000/LConn2 -- _CN_178968761_400000_CN_98218556_400000/LConn2 -- _CN_178968761_400000_CN_418832515_400000/LConn2 -- L_178968761/LConn2
  _CN_185497473_400000_CN_178968761_400000/RConn3 -- T_178968761_765000;400000_/RConn3 -- _CN_98231311_400000_CN_178968761_400000/LConn3 -- _CN_179140081_400000_CN_178968761_400000/LConn3 -- _CN_65600948_400000_CN_178968761_400000/LConn3 -- _CN_178968761_400000_CN_98218556_400000/LConn3 -- _CN_178968761_400000_CN_418832515_400000/LConn3 -- L_178968761/LConn3 -- bus182/LConn1
  _CN_185497473_400000_CN_75136015_400000/RConn1 -- T_75136015_400000;275000_Minerva_Substation/LConn1 -- _CN_75136015_400000_CN_87404898_400000/LConn1 -- _CN_75136015_400000_CN_83525879_400000/RConn1 -- _CN_178882935_400000_CN_75136015_400000/LConn1 -- _CN_185171518_400000_CN_75136015_400000/LConn1
  _CN_185497473_400000_CN_75136015_400000/RConn2 -- T_75136015_400000;275000_Minerva_Substation/LConn2 -- _CN_75136015_400000_CN_87404898_400000/LConn2 -- _CN_75136015_400000_CN_83525879_400000/RConn2 -- _CN_178882935_400000_CN_75136015_400000/LConn2 -- _CN_185171518_400000_CN_75136015_400000/LConn2
  _CN_185497473_400000_CN_75136015_400000/RConn3 -- T_75136015_400000;275000_Minerva_Substation/LConn3 -- _CN_75136015_400000_CN_87404898_400000/LConn3 -- bus183/LConn1 -- _CN_75136015_400000_CN_83525879_400000/RConn3 -- _CN_178882935_400000_CN_75136015_400000/LConn3 -- _CN_185171518_400000_CN_75136015_400000/LConn3
  _CN_92348290_400000_CN_181366662_400000/LConn1 -- T_92348290_400000;275000_Perseus_Substation/RConn1 -- _CN_92348290_400000_CN_386388564_400000/LConn1 -- _CN_92348290_400000_CN_142414070_400000/LConn1
  _CN_92348290_400000_CN_181366662_400000/LConn2 -- T_92348290_400000;275000_Perseus_Substation/RConn2 -- _CN_92348290_400000_CN_386388564_400000/LConn2 -- _CN_92348290_400000_CN_142414070_400000/LConn2
  _CN_92348290_400000_CN_181366662_400000/LConn3 -- T_92348290_400000;275000_Perseus_Substation/RConn3 -- _CN_92348290_400000_CN_386388564_400000/LConn3 -- bus184/LConn1 -- _CN_92348290_400000_CN_142414070_400000/LConn3
  _CN_92348290_400000_CN_181366662_400000/RConn1 -- T_181366662_400000_Beta_Substation/RConn1 -- _CN_181366662_400000_CN_142414070_400000/LConn1 -- L_181366662/LConn1
  _CN_92348290_400000_CN_181366662_400000/RConn2 -- T_181366662_400000_Beta_Substation/RConn2 -- _CN_181366662_400000_CN_142414070_400000/LConn2 -- L_181366662/LConn2
  _CN_92348290_400000_CN_181366662_400000/RConn3 -- T_181366662_400000_Beta_Substation/RConn3 -- _CN_181366662_400000_CN_142414070_400000/LConn3 -- L_181366662/LConn3 -- bus185/LConn1
  _CN_92348290_400000_CN_142414070_400000/RConn1 -- T_142414070_400000_Hydra_Substation/LConn1 -- _CN_181366662_400000_CN_142414070_400000/RConn1 -- _CN_167590549_400000_CN_142414070_400000/LConn1 -- _CN_183402339_400000_CN_142414070_400000/LConn1 -- _CN_89173873_400000_CN_142414070_400000/LConn1 -- _CN_142414070_400000_CN_89637370_400000/LConn1
  _CN_92348290_400000_CN_142414070_400000/RConn2 -- T_142414070_400000_Hydra_Substation/LConn2 -- _CN_181366662_400000_CN_142414070_400000/RConn2 -- _CN_167590549_400000_CN_142414070_400000/LConn2 -- _CN_183402339_400000_CN_142414070_400000/LConn2 -- _CN_89173873_400000_CN_142414070_400000/LConn2 -- _CN_142414070_400000_CN_89637370_400000/LConn2
  _CN_92348290_400000_CN_142414070_400000/RConn3 -- T_142414070_400000_Hydra_Substation/LConn3 -- _CN_181366662_400000_CN_142414070_400000/RConn3 -- _CN_167590549_400000_CN_142414070_400000/LConn3 -- _CN_183402339_400000_CN_142414070_400000/LConn3 -- _CN_89173873_400000_CN_142414070_400000/LConn3 -- _CN_142414070_400000_CN_89637370_400000/LConn3 -- bus186/LConn1
  _CN_92348290_400000_CN_386388564_400000/RConn1 -- T_386388564__/LConn1 -- _CN_98231311_400000_CN_386388564_400000/LConn1 -- _CN_386388564_400000_CN_418832515_400000/LConn1
  _CN_92348290_400000_CN_386388564_400000/RConn2 -- T_386388564__/LConn2 -- _CN_98231311_400000_CN_386388564_400000/LConn2 -- _CN_386388564_400000_CN_418832515_400000/LConn2
  _CN_92348290_400000_CN_386388564_400000/RConn3 -- T_386388564__/LConn3 -- _CN_98231311_400000_CN_386388564_400000/LConn3 -- _CN_386388564_400000_CN_418832515_400000/LConn3 -- bus187/LConn1
  T_184560833__/LConn1 -- _CN_184560833_400000_CN_185171511_400000/RConn1
  T_184560833__/LConn2 -- _CN_184560833_400000_CN_185171511_400000/RConn2
  _CN_184560833_400000_CN_185171511_400000/RConn3 -- T_184560833__/LConn3 -- bus188/LConn1
  _CN_209365700_400000_CN_418832512_400000/LConn1 -- T_209365700_400000_/LConn1 -- _CN_209365700_400000_CN_167648085_400000/LConn1 -- _CN_209365700_400000_CN_179136373_400000/LConn1 -- _CN_209365700_400000_CN_183775937_400000/LConn1
  _CN_209365700_400000_CN_418832512_400000/LConn2 -- T_209365700_400000_/LConn2 -- _CN_209365700_400000_CN_167648085_400000/LConn2 -- _CN_209365700_400000_CN_179136373_400000/LConn2 -- _CN_209365700_400000_CN_183775937_400000/LConn2
  _CN_209365700_400000_CN_418832512_400000/LConn3 -- T_209365700_400000_/LConn3 -- _CN_209365700_400000_CN_167648085_400000/LConn3 -- _CN_209365700_400000_CN_179136373_400000/LConn3 -- _CN_209365700_400000_CN_183775937_400000/LConn3 -- bus189/LConn1
  _CN_209365700_400000_CN_418832512_400000/RConn1 -- G_418832512_Camden_Power_Station/RConn1 -- _CN_183757901_400000_CN_418832512_400000/LConn1 -- _CN_104080393_400000_CN_418832512_400000/LConn1 -- _CN_238322344_400000_CN_418832512_400000/LConn1
  _CN_209365700_400000_CN_418832512_400000/RConn2 -- G_418832512_Camden_Power_Station/RConn2 -- _CN_183757901_400000_CN_418832512_400000/LConn2 -- _CN_104080393_400000_CN_418832512_400000/LConn2 -- _CN_238322344_400000_CN_418832512_400000/LConn2
  _CN_209365700_400000_CN_418832512_400000/RConn3 -- G_418832512_Camden_Power_Station/RConn3 -- _CN_183757901_400000_CN_418832512_400000/LConn3 -- bus190/LConn1 -- _CN_104080393_400000_CN_418832512_400000/LConn3 -- _CN_238322344_400000_CN_418832512_400000/LConn3
  _CN_209365700_400000_CN_167648085_400000/RConn1 -- T_167648085__/LConn1 -- _CN_219596295_400000_CN_167648085_400000/LConn1 -- _CN_183759046_400000_CN_167648085_400000/LConn1 -- _CN_181284049_400000_CN_167648085_400000/LConn1 -- _CN_167648085_400000_CN_183775937_400000/LConn1 -- _CN_105759402_400000_CN_167648085_400000/LConn1
  _CN_209365700_400000_CN_167648085_400000/RConn2 -- T_167648085__/LConn2 -- _CN_219596295_400000_CN_167648085_400000/LConn2 -- _CN_183759046_400000_CN_167648085_400000/LConn2 -- _CN_181284049_400000_CN_167648085_400000/LConn2 -- _CN_167648085_400000_CN_183775937_400000/LConn2 -- _CN_105759402_400000_CN_167648085_400000/LConn2
  _CN_209365700_400000_CN_167648085_400000/RConn3 -- T_167648085__/LConn3 -- _CN_219596295_400000_CN_167648085_400000/LConn3 -- _CN_183759046_400000_CN_167648085_400000/LConn3 -- _CN_181284049_400000_CN_167648085_400000/LConn3 -- _CN_167648085_400000_CN_183775937_400000/LConn3 -- bus191/LConn1 -- _CN_105759402_400000_CN_167648085_400000/LConn3
  _CN_209365700_400000_CN_179136373_400000/RConn1 -- T_179136373__/RConn1 -- _CN_179136373_400000_CN_183775937_400000/LConn1 -- L_179136373/LConn1
  _CN_209365700_400000_CN_179136373_400000/RConn2 -- T_179136373__/RConn2 -- _CN_179136373_400000_CN_183775937_400000/LConn2 -- L_179136373/LConn2
  _CN_209365700_400000_CN_179136373_400000/RConn3 -- T_179136373__/RConn3 -- _CN_179136373_400000_CN_183775937_400000/LConn3 -- L_179136373/LConn3 -- bus192/LConn1
  _CN_209365700_400000_CN_183775937_400000/RConn1 -- G_183775937_Majuba_Power_Station/RConn1 -- _CN_127585817_400000_CN_183775937_400000/LConn1 -- _CN_167648085_400000_CN_183775937_400000/RConn1 -- _CN_179136373_400000_CN_183775937_400000/RConn1
  _CN_209365700_400000_CN_183775937_400000/RConn2 -- G_183775937_Majuba_Power_Station/RConn2 -- _CN_127585817_400000_CN_183775937_400000/LConn2 -- _CN_167648085_400000_CN_183775937_400000/RConn2 -- _CN_179136373_400000_CN_183775937_400000/RConn2
  _CN_209365700_400000_CN_183775937_400000/RConn3 -- G_183775937_Majuba_Power_Station/RConn3 -- _CN_127585817_400000_CN_183775937_400000/LConn3 -- _CN_167648085_400000_CN_183775937_400000/RConn3 -- _CN_179136373_400000_CN_183775937_400000/RConn3 -- bus193/LConn1
  _CN_104080393_400000_CN_418832512_400000/RConn1 -- T_104080393__/LConn1 -- _CN_104080393_400000_CN_183759046_400000/LConn1
  _CN_104080393_400000_CN_418832512_400000/RConn2 -- T_104080393__/LConn2 -- _CN_104080393_400000_CN_183759046_400000/LConn2
  _CN_104080393_400000_CN_418832512_400000/RConn3 -- T_104080393__/LConn3 -- _CN_104080393_400000_CN_183759046_400000/LConn3 -- bus194/LConn1
  _CN_104080393_400000_CN_183759046_400000/RConn1 -- T_183759046__/LConn1 -- _CN_183759046_400000_CN_167648085_400000/RConn1 -- _CN_183759046_400000_CN_181284049_400000/LConn1
  _CN_104080393_400000_CN_183759046_400000/RConn2 -- T_183759046__/LConn2 -- _CN_183759046_400000_CN_167648085_400000/RConn2 -- _CN_183759046_400000_CN_181284049_400000/LConn2
  _CN_104080393_400000_CN_183759046_400000/RConn3 -- T_183759046__/LConn3 -- _CN_183759046_400000_CN_167648085_400000/RConn3 -- _CN_183759046_400000_CN_181284049_400000/LConn3 -- bus195/LConn1
  _CN_230551819_400000_CN_182408147_400000/RConn1 -- T_182408147__/LConn1 -- _CN_182408147_400000_CN_184552955_400000/LConn1 -- _CN_182408147_400000_CN_87404898_400000/LConn1 -- _CN_87434264_400000_CN_182408147_400000/LConn1 -- _CN_184201271_400000_CN_182408147_400000/LConn1
  _CN_230551819_400000_CN_182408147_400000/RConn2 -- T_182408147__/LConn2 -- _CN_182408147_400000_CN_184552955_400000/LConn2 -- _CN_182408147_400000_CN_87404898_400000/LConn2 -- _CN_87434264_400000_CN_182408147_400000/LConn2 -- _CN_184201271_400000_CN_182408147_400000/LConn2
  _CN_230551819_400000_CN_182408147_400000/RConn3 -- T_182408147__/LConn3 -- _CN_182408147_400000_CN_184552955_400000/LConn3 -- _CN_182408147_400000_CN_87404898_400000/LConn3 -- bus196/LConn1 -- _CN_87434264_400000_CN_182408147_400000/LConn3 -- _CN_184201271_400000_CN_182408147_400000/LConn3
  _CN_98231311_400000_CN_386388564_400000/RConn1 -- T_98231311_400000_Grootvlei_Substation/LConn1 -- _CN_98231311_400000_CN_178968761_400000/RConn1
  _CN_98231311_400000_CN_386388564_400000/RConn2 -- T_98231311_400000_Grootvlei_Substation/LConn2 -- _CN_98231311_400000_CN_178968761_400000/RConn2
  _CN_98231311_400000_CN_386388564_400000/RConn3 -- T_98231311_400000_Grootvlei_Substation/LConn3 -- _CN_98231311_400000_CN_178968761_400000/RConn3 -- bus197/LConn1
  _CN_156418705_400000_CN_418832508_275000/RConn1 -- T_156418705__/LConn1 -- _CN_156418705_400000_CN_184552955_400000/LConn1
  _CN_156418705_400000_CN_418832508_275000/RConn2 -- T_156418705__/LConn2 -- _CN_156418705_400000_CN_184552955_400000/LConn2
  _CN_156418705_400000_CN_418832508_275000/RConn3 -- T_156418705__/LConn3 -- _CN_156418705_400000_CN_184552955_400000/LConn3 -- bus198/LConn1
  _CN_156418705_400000_CN_184552955_400000/RConn1 -- T_184552955__/LConn1 -- _CN_182408147_400000_CN_184552955_400000/RConn1
  _CN_156418705_400000_CN_184552955_400000/RConn2 -- T_184552955__/LConn2 -- _CN_182408147_400000_CN_184552955_400000/RConn2
  _CN_156418705_400000_CN_184552955_400000/RConn3 -- T_184552955__/LConn3 -- _CN_182408147_400000_CN_184552955_400000/RConn3 -- bus199/LConn1
  _CN_167590549_400000_CN_89173873_400000/LConn1 -- T_167590549_400000_Droërivier_Substation/LConn1 -- _CN_167590549_400000_CN_142414070_400000/RConn1
  _CN_167590549_400000_CN_89173873_400000/LConn2 -- T_167590549_400000_Droërivier_Substation/LConn2 -- _CN_167590549_400000_CN_142414070_400000/RConn2
  _CN_167590549_400000_CN_89173873_400000/LConn3 -- T_167590549_400000_Droërivier_Substation/LConn3 -- _CN_167590549_400000_CN_142414070_400000/RConn3 -- bus200/LConn1
  _CN_167590549_400000_CN_89173873_400000/RConn1 -- T_89173873__/LConn1 -- _CN_89173873_400000_CN_142414070_400000/RConn1
  _CN_167590549_400000_CN_89173873_400000/RConn2 -- T_89173873__/LConn2 -- _CN_89173873_400000_CN_142414070_400000/RConn2
  _CN_167590549_400000_CN_89173873_400000/RConn3 -- T_89173873__/LConn3 -- _CN_89173873_400000_CN_142414070_400000/RConn3 -- bus201/LConn1
  _CN_87434264_400000_CN_184201271_400000/LConn1 -- T_87434264_400000_/LConn1 -- _CN_87434264_400000_CN_178240542_400000/LConn1 -- _CN_87434264_400000_CN_87404898_400000/LConn1 -- _CN_87434264_400000_CN_167540668_400000/LConn1 -- _CN_87434264_400000_CN_182408147_400000/RConn1
  _CN_87434264_400000_CN_184201271_400000/LConn2 -- T_87434264_400000_/LConn2 -- _CN_87434264_400000_CN_178240542_400000/LConn2 -- _CN_87434264_400000_CN_87404898_400000/LConn2 -- _CN_87434264_400000_CN_167540668_400000/LConn2 -- _CN_87434264_400000_CN_182408147_400000/RConn2
  _CN_87434264_400000_CN_184201271_400000/LConn3 -- T_87434264_400000_/LConn3 -- _CN_87434264_400000_CN_178240542_400000/LConn3 -- bus202/LConn1 -- _CN_87434264_400000_CN_87404898_400000/LConn3 -- _CN_87434264_400000_CN_167540668_400000/LConn3 -- _CN_87434264_400000_CN_182408147_400000/RConn3
  _CN_87434264_400000_CN_184201271_400000/RConn1 -- T_184201271__/LConn1 -- _CN_184201271_400000_CN_182408147_400000/RConn1
  _CN_87434264_400000_CN_184201271_400000/RConn2 -- T_184201271__/LConn2 -- _CN_184201271_400000_CN_182408147_400000/RConn2
  _CN_87434264_400000_CN_184201271_400000/RConn3 -- T_184201271__/LConn3 -- _CN_184201271_400000_CN_182408147_400000/RConn3 -- bus203/LConn1
  _CN_87434264_400000_CN_87404898_400000/RConn1 -- T_87404898_400000;275000_Pluto_Substation/LConn1 -- _CN_178882935_400000_CN_87404898_400000/LConn1 -- _CN_182408147_400000_CN_87404898_400000/RConn1 -- _CN_75136015_400000_CN_87404898_400000/RConn1 -- _CN_103079596_400000_CN_87404898_400000/LConn1
  _CN_87434264_400000_CN_87404898_400000/RConn2 -- T_87404898_400000;275000_Pluto_Substation/LConn2 -- _CN_178882935_400000_CN_87404898_400000/LConn2 -- _CN_182408147_400000_CN_87404898_400000/RConn2 -- _CN_75136015_400000_CN_87404898_400000/RConn2 -- _CN_103079596_400000_CN_87404898_400000/LConn2
  _CN_87434264_400000_CN_87404898_400000/RConn3 -- T_87404898_400000;275000_Pluto_Substation/LConn3 -- _CN_178882935_400000_CN_87404898_400000/LConn3 -- _CN_182408147_400000_CN_87404898_400000/RConn3 -- _CN_75136015_400000_CN_87404898_400000/RConn3 -- bus204/LConn1 -- _CN_103079596_400000_CN_87404898_400000/LConn3
  _CN_87434264_400000_CN_167540668_400000/RConn1 -- T_167540668_400000_/RConn1 -- _CN_103079596_400000_CN_167540668_400000/LConn1 -- L_167540668/LConn1
  _CN_87434264_400000_CN_167540668_400000/RConn2 -- T_167540668_400000_/RConn2 -- _CN_103079596_400000_CN_167540668_400000/LConn2 -- L_167540668/LConn2
  _CN_87434264_400000_CN_167540668_400000/RConn3 -- T_167540668_400000_/RConn3 -- _CN_103079596_400000_CN_167540668_400000/LConn3 -- L_167540668/LConn3 -- bus205/LConn1
  _CN_87434264_400000_CN_178240542_400000/RConn1 -- T_178240542__/LConn1 -- _CN_178240542_400000_CN_105811523_400000/LConn1
  _CN_87434264_400000_CN_178240542_400000/RConn2 -- T_178240542__/LConn2 -- _CN_178240542_400000_CN_105811523_400000/LConn2
  _CN_87434264_400000_CN_178240542_400000/RConn3 -- T_178240542__/LConn3 -- _CN_178240542_400000_CN_105811523_400000/LConn3 -- bus206/LConn1
  _CN_127585817_400000_CN_183775937_400000/RConn1 -- T_127585817__/LConn1 -- _CN_127585817_400000_CN_105759402_400000/LConn1 -- _CN_127585817_400000_CN_181284049_400000/LConn1 -- _CN_127585817_400000_CN_176362710_400000/LConn1
  _CN_127585817_400000_CN_183775937_400000/RConn2 -- T_127585817__/LConn2 -- _CN_127585817_400000_CN_105759402_400000/LConn2 -- _CN_127585817_400000_CN_181284049_400000/LConn2 -- _CN_127585817_400000_CN_176362710_400000/LConn2
  _CN_127585817_400000_CN_183775937_400000/RConn3 -- T_127585817__/LConn3 -- _CN_127585817_400000_CN_105759402_400000/LConn3 -- bus207/LConn1 -- _CN_127585817_400000_CN_181284049_400000/LConn3 -- _CN_127585817_400000_CN_176362710_400000/LConn3
  _CN_127585817_400000_CN_181284049_400000/RConn1 -- T_181284049__/LConn1 -- _CN_107391770_400000_CN_181284049_400000/LConn1 -- _CN_183759046_400000_CN_181284049_400000/RConn1 -- _CN_181284049_400000_CN_167648085_400000/RConn1
  _CN_127585817_400000_CN_181284049_400000/RConn2 -- T_181284049__/LConn2 -- _CN_107391770_400000_CN_181284049_400000/LConn2 -- _CN_183759046_400000_CN_181284049_400000/RConn2 -- _CN_181284049_400000_CN_167648085_400000/RConn2
  _CN_127585817_400000_CN_181284049_400000/RConn3 -- T_181284049__/LConn3 -- _CN_107391770_400000_CN_181284049_400000/LConn3 -- _CN_183759046_400000_CN_181284049_400000/RConn3 -- _CN_181284049_400000_CN_167648085_400000/RConn3 -- bus208/LConn1
  _CN_127585817_400000_CN_176362710_400000/RConn1 -- T_176362710__/LConn1 -- _CN_107391770_400000_CN_176362710_400000/LConn1 -- _CN_207991752_400000_CN_176362710_400000/LConn1
  _CN_127585817_400000_CN_176362710_400000/RConn2 -- T_176362710__/LConn2 -- _CN_107391770_400000_CN_176362710_400000/LConn2 -- _CN_207991752_400000_CN_176362710_400000/LConn2
  _CN_127585817_400000_CN_176362710_400000/RConn3 -- T_176362710__/LConn3 -- _CN_107391770_400000_CN_176362710_400000/LConn3 -- _CN_207991752_400000_CN_176362710_400000/LConn3 -- bus209/LConn1
  _CN_127585817_400000_CN_105759402_400000/RConn1 -- T_105759402__/LConn1 -- _CN_105759402_400000_CN_167648085_400000/RConn1
  _CN_127585817_400000_CN_105759402_400000/RConn2 -- T_105759402__/LConn2 -- _CN_105759402_400000_CN_167648085_400000/RConn2
  _CN_127585817_400000_CN_105759402_400000/RConn3 -- T_105759402__/LConn3 -- _CN_105759402_400000_CN_167648085_400000/RConn3 -- bus210/LConn1
  _CN_107391770_400000_CN_176362710_400000/RConn1 -- T_107391770_400000;275000_/LConn1 -- _CN_107391770_400000_CN_181284049_400000/RConn1
  _CN_107391770_400000_CN_176362710_400000/RConn2 -- T_107391770_400000;275000_/LConn2 -- _CN_107391770_400000_CN_181284049_400000/RConn2
  _CN_107391770_400000_CN_176362710_400000/RConn3 -- T_107391770_400000;275000_/LConn3 -- _CN_107391770_400000_CN_181284049_400000/RConn3 -- bus211/LConn1
  _CN_62191005_400000_CN_252396496_132000/RConn1 -- T_62191005_400000;132000_Muldersvlei_Substation/LConn1 -- _CN_62191005_400000_CN_62193952_400000/LConn1 -- _CN_62191005_400000_CN_120584910_400000/LConn1 -- _CN_62191005_400000_CN_219384657_400000/LConn1 -- _CN_62191005_400000_CN_177800991_400000/LConn1
  _CN_62191005_400000_CN_252396496_132000/RConn2 -- T_62191005_400000;132000_Muldersvlei_Substation/LConn2 -- _CN_62191005_400000_CN_62193952_400000/LConn2 -- _CN_62191005_400000_CN_120584910_400000/LConn2 -- _CN_62191005_400000_CN_219384657_400000/LConn2 -- _CN_62191005_400000_CN_177800991_400000/LConn2
  _CN_62191005_400000_CN_252396496_132000/RConn3 -- T_62191005_400000;132000_Muldersvlei_Substation/LConn3 -- _CN_62191005_400000_CN_62193952_400000/LConn3 -- _CN_62191005_400000_CN_120584910_400000/LConn3 -- _CN_62191005_400000_CN_219384657_400000/LConn3 -- bus212/LConn1 -- _CN_62191005_400000_CN_177800991_400000/LConn3
  _CN_62191005_400000_CN_177800991_400000/RConn1 -- T_177800991_400000;132000_Bacchus_Substation/LConn1 -- _CN_177800991_400000_CN_121995134_400000/LConn1 -- _CN_177800991_400000_CN_418863864_400000/LConn1
  _CN_62191005_400000_CN_177800991_400000/RConn2 -- T_177800991_400000;132000_Bacchus_Substation/LConn2 -- _CN_177800991_400000_CN_121995134_400000/LConn2 -- _CN_177800991_400000_CN_418863864_400000/LConn2
  _CN_62191005_400000_CN_177800991_400000/RConn3 -- T_177800991_400000;132000_Bacchus_Substation/LConn3 -- _CN_177800991_400000_CN_121995134_400000/LConn3 -- bus213/LConn1 -- _CN_177800991_400000_CN_418863864_400000/LConn3
  _CN_62191005_400000_CN_62193952_400000/RConn1 -- T_62193952_400000;132000_Acacia_Park_Substation/LConn1 -- _CN_62193952_400000_CN_62218063_400000/LConn1 -- _CN_62193952_400000_CN_252396496_132000/RConn1
  _CN_62191005_400000_CN_62193952_400000/RConn2 -- T_62193952_400000;132000_Acacia_Park_Substation/LConn2 -- _CN_62193952_400000_CN_62218063_400000/LConn2 -- _CN_62193952_400000_CN_252396496_132000/RConn2
  _CN_62191005_400000_CN_62193952_400000/RConn3 -- T_62193952_400000;132000_Acacia_Park_Substation/LConn3 -- _CN_62193952_400000_CN_62218063_400000/LConn3 -- _CN_62193952_400000_CN_252396496_132000/RConn3 -- bus214/LConn1
  _CN_62191005_400000_CN_120584910_400000/RConn1 -- T_120584910_400000;132000_Stikland_Substation/LConn1 -- _CN_102682082_400000_CN_120584910_400000/LConn1
  _CN_62191005_400000_CN_120584910_400000/RConn2 -- T_120584910_400000;132000_Stikland_Substation/LConn2 -- _CN_102682082_400000_CN_120584910_400000/LConn2
  _CN_62191005_400000_CN_120584910_400000/RConn3 -- T_120584910_400000;132000_Stikland_Substation/LConn3 -- _CN_102682082_400000_CN_120584910_400000/LConn3 -- bus215/LConn1
  _CN_62191005_400000_CN_219384657_400000/RConn1 -- T_219384657__Omega_Substation/LConn1 -- _CN_219384657_400000_CN_252396496_132000/RConn1
  _CN_62191005_400000_CN_219384657_400000/RConn2 -- T_219384657__Omega_Substation/LConn2 -- _CN_219384657_400000_CN_252396496_132000/RConn2
  _CN_62191005_400000_CN_219384657_400000/RConn3 -- T_219384657__Omega_Substation/LConn3 -- _CN_219384657_400000_CN_252396496_132000/RConn3 -- bus216/LConn1
  _CN_178240542_400000_CN_105811523_400000/RConn1 -- T_105811523_400000;275000_Glockner_Substation/LConn1 -- _CN_65600948_400000_CN_105811523_400000/LConn1 -- _CN_105811523_400000_CN_418832515_400000/LConn1
  _CN_178240542_400000_CN_105811523_400000/RConn2 -- T_105811523_400000;275000_Glockner_Substation/LConn2 -- _CN_65600948_400000_CN_105811523_400000/LConn2 -- _CN_105811523_400000_CN_418832515_400000/LConn2
  _CN_178240542_400000_CN_105811523_400000/RConn3 -- T_105811523_400000;275000_Glockner_Substation/LConn3 -- _CN_65600948_400000_CN_105811523_400000/LConn3 -- _CN_105811523_400000_CN_418832515_400000/LConn3 -- bus217/LConn1
  G_418863864_Palmiet_Pumped_Storage_Scheme/RConn1 -- _CN_177800991_400000_CN_418863864_400000/RConn1
  G_418863864_Palmiet_Pumped_Storage_Scheme/RConn2 -- _CN_177800991_400000_CN_418863864_400000/RConn2
  _CN_177800991_400000_CN_418863864_400000/RConn3 -- G_418863864_Palmiet_Pumped_Storage_Scheme/RConn3 -- bus218/LConn1
  _CN_177800991_400000_CN_121995134_400000/RConn1 -- T_121995134_400000_Proteus/LConn1 -- _CN_169789536_400000_CN_121995134_400000/LConn1
  _CN_177800991_400000_CN_121995134_400000/RConn2 -- T_121995134_400000_Proteus/LConn2 -- _CN_169789536_400000_CN_121995134_400000/LConn2
  _CN_177800991_400000_CN_121995134_400000/RConn3 -- T_121995134_400000_Proteus/LConn3 -- _CN_169789536_400000_CN_121995134_400000/LConn3 -- bus219/LConn1
  T_62218063_400000_Philippi_Substation/LConn1 -- _CN_62193952_400000_CN_62218063_400000/RConn1
  T_62218063_400000_Philippi_Substation/LConn2 -- _CN_62193952_400000_CN_62218063_400000/RConn2
  _CN_62193952_400000_CN_62218063_400000/RConn3 -- T_62218063_400000_Philippi_Substation/LConn3 -- bus220/LConn1
  T_131625968_132000_Nseleni_Substation/LConn1 -- _CN_131625968_400000_CN_219596295_400000/LConn1
  T_131625968_132000_Nseleni_Substation/LConn2 -- _CN_131625968_400000_CN_219596295_400000/LConn2
  _CN_131625968_400000_CN_219596295_400000/LConn3 -- T_131625968_132000_Nseleni_Substation/LConn3 -- bus221/LConn1
  _CN_131625968_400000_CN_219596295_400000/RConn1 -- T_219596295__/LConn1 -- _CN_219596295_400000_CN_183757901_400000/LConn1 -- _CN_219596295_400000_CN_167648085_400000/RConn1
  _CN_131625968_400000_CN_219596295_400000/RConn2 -- T_219596295__/LConn2 -- _CN_219596295_400000_CN_183757901_400000/LConn2 -- _CN_219596295_400000_CN_167648085_400000/RConn2
  _CN_131625968_400000_CN_219596295_400000/RConn3 -- T_219596295__/LConn3 -- _CN_219596295_400000_CN_183757901_400000/LConn3 -- _CN_219596295_400000_CN_167648085_400000/RConn3 -- bus222/LConn1
  T_169647963_400000;220000_Grassridge_Substation/LConn1 -- _CN_169647963_400000_CN_90454383_400000/LConn1
  T_169647963_400000;220000_Grassridge_Substation/LConn2 -- _CN_169647963_400000_CN_90454383_400000/LConn2
  _CN_169647963_400000_CN_90454383_400000/LConn3 -- T_169647963_400000;220000_Grassridge_Substation/LConn3 -- bus223/LConn1
  _CN_169647963_400000_CN_90454383_400000/RConn1 -- T_90454383_400000;220000_Grassridge_Substation/LConn1 -- _CN_90454383_400000_CN_89637370_400000/LConn1
  _CN_169647963_400000_CN_90454383_400000/RConn2 -- T_90454383_400000;220000_Grassridge_Substation/LConn2 -- _CN_90454383_400000_CN_89637370_400000/LConn2
  _CN_169647963_400000_CN_90454383_400000/RConn3 -- T_90454383_400000;220000_Grassridge_Substation/LConn3 -- _CN_90454383_400000_CN_89637370_400000/LConn3 -- bus224/LConn1
  _CN_179140081_400000_CN_98218556_400000/LConn1 -- T_179140081_400000_/LConn1 -- _CN_179140081_400000_CN_178968761_400000/RConn1
  _CN_179140081_400000_CN_98218556_400000/LConn2 -- T_179140081_400000_/LConn2 -- _CN_179140081_400000_CN_178968761_400000/RConn2
  _CN_179140081_400000_CN_98218556_400000/LConn3 -- T_179140081_400000_/LConn3 -- _CN_179140081_400000_CN_178968761_400000/RConn3 -- bus225/LConn1
  _CN_179140081_400000_CN_98218556_400000/RConn1 -- T_98218556__/LConn1 -- _CN_178968761_400000_CN_98218556_400000/RConn1 -- _CN_98218556_400000_CN_185341297_400000/LConn1
  _CN_179140081_400000_CN_98218556_400000/RConn2 -- T_98218556__/LConn2 -- _CN_178968761_400000_CN_98218556_400000/RConn2 -- _CN_98218556_400000_CN_185341297_400000/LConn2
  _CN_179140081_400000_CN_98218556_400000/RConn3 -- T_98218556__/LConn3 -- _CN_178968761_400000_CN_98218556_400000/RConn3 -- _CN_98218556_400000_CN_185341297_400000/LConn3 -- bus226/LConn1
  _CN_238322344_400000_CN_418832512_400000/RConn1 -- T_238322344__/LConn1 -- _CN_238322344_400000_CN_185171511_400000/RConn1
  _CN_238322344_400000_CN_418832512_400000/RConn2 -- T_238322344__/LConn2 -- _CN_238322344_400000_CN_185171511_400000/RConn2
  _CN_238322344_400000_CN_418832512_400000/RConn3 -- T_238322344__/LConn3 -- _CN_238322344_400000_CN_185171511_400000/RConn3 -- bus227/LConn1
  _CN_219596295_400000_CN_183757901_400000/RConn1 -- T_183757901__Normandie_Substation/LConn1 -- _CN_183757901_400000_CN_418832512_400000/RConn1
  _CN_219596295_400000_CN_183757901_400000/RConn2 -- T_183757901__Normandie_Substation/LConn2 -- _CN_183757901_400000_CN_418832512_400000/RConn2
  _CN_219596295_400000_CN_183757901_400000/RConn3 -- T_183757901__Normandie_Substation/LConn3 -- _CN_183757901_400000_CN_418832512_400000/RConn3 -- bus228/LConn1
  _CN_103079596_400000_CN_87404898_400000/RConn1 -- T_103079596__/LConn1 -- _CN_103079596_400000_CN_167540668_400000/RConn1
  _CN_103079596_400000_CN_87404898_400000/RConn2 -- T_103079596__/LConn2 -- _CN_103079596_400000_CN_167540668_400000/RConn2
  _CN_103079596_400000_CN_87404898_400000/RConn3 -- T_103079596__/LConn3 -- _CN_103079596_400000_CN_167540668_400000/RConn3 -- bus229/LConn1
  _CN_170672051_400000_CN_83525879_400000/RConn1 -- T_170672051__/LConn1 -- _CN_170672051_400000_CN_185171511_400000/RConn1 -- _CN_170672051_400000_CN_418832508_275000/RConn1 -- _CN_170672051_400000_CN_185341297_400000/LConn1
  _CN_170672051_400000_CN_83525879_400000/RConn2 -- T_170672051__/LConn2 -- _CN_170672051_400000_CN_185171511_400000/RConn2 -- _CN_170672051_400000_CN_418832508_275000/RConn2 -- _CN_170672051_400000_CN_185341297_400000/LConn2
  _CN_170672051_400000_CN_83525879_400000/RConn3 -- T_170672051__/LConn3 -- _CN_170672051_400000_CN_185171511_400000/RConn3 -- _CN_170672051_400000_CN_418832508_275000/RConn3 -- _CN_170672051_400000_CN_185341297_400000/LConn3 -- bus230/LConn1
  _CN_170672051_400000_CN_185341297_400000/RConn1 -- G_185341297_Hendrina_Power_Station/RConn1 -- _CN_98218556_400000_CN_185341297_400000/RConn1 -- _CN_220129604_400000_CN_185341297_400000/LConn1
  _CN_170672051_400000_CN_185341297_400000/RConn2 -- G_185341297_Hendrina_Power_Station/RConn2 -- _CN_98218556_400000_CN_185341297_400000/RConn2 -- _CN_220129604_400000_CN_185341297_400000/LConn2
  _CN_170672051_400000_CN_185341297_400000/RConn3 -- G_185341297_Hendrina_Power_Station/RConn3 -- _CN_98218556_400000_CN_185341297_400000/RConn3 -- _CN_220129604_400000_CN_185341297_400000/LConn3 -- bus231/LConn1
  _CN_65600948_400000_CN_178968761_400000/RConn1 -- T_65600948__/LConn1 -- _CN_65600948_400000_CN_105811523_400000/RConn1 -- _CN_65600948_400000_CN_185171511_400000/RConn1 -- _CN_65600948_400000_CN_418832515_400000/LConn1
  _CN_65600948_400000_CN_178968761_400000/RConn2 -- T_65600948__/LConn2 -- _CN_65600948_400000_CN_105811523_400000/RConn2 -- _CN_65600948_400000_CN_185171511_400000/RConn2 -- _CN_65600948_400000_CN_418832515_400000/LConn2
  _CN_65600948_400000_CN_178968761_400000/RConn3 -- T_65600948__/LConn3 -- _CN_65600948_400000_CN_105811523_400000/RConn3 -- _CN_65600948_400000_CN_185171511_400000/RConn3 -- _CN_65600948_400000_CN_418832515_400000/LConn3 -- bus232/LConn1
  _CN_65600948_400000_CN_418832515_400000/RConn1 -- G_418832515_Grootvlei_Power_Station/RConn1 -- _CN_105811523_400000_CN_418832515_400000/RConn1 -- _CN_386388564_400000_CN_418832515_400000/RConn1 -- _CN_178968761_400000_CN_418832515_400000/RConn1
  _CN_65600948_400000_CN_418832515_400000/RConn2 -- G_418832515_Grootvlei_Power_Station/RConn2 -- _CN_105811523_400000_CN_418832515_400000/RConn2 -- _CN_386388564_400000_CN_418832515_400000/RConn2 -- _CN_178968761_400000_CN_418832515_400000/RConn2
  _CN_65600948_400000_CN_418832515_400000/RConn3 -- G_418832515_Grootvlei_Power_Station/RConn3 -- _CN_105811523_400000_CN_418832515_400000/RConn3 -- _CN_386388564_400000_CN_418832515_400000/RConn3 -- bus233/LConn1 -- _CN_178968761_400000_CN_418832515_400000/RConn3
  T_183212853_400000_Neptune_Main_Transmission_Substation/LConn1 -- _CN_183212853_400000_CN_107937167_400000/LConn1
  T_183212853_400000_Neptune_Main_Transmission_Substation/LConn2 -- _CN_183212853_400000_CN_107937167_400000/LConn2
  _CN_183212853_400000_CN_107937167_400000/LConn3 -- T_183212853_400000_Neptune_Main_Transmission_Substation/LConn3 -- bus234/LConn1
  T_107937167_400000_Delphi_Substation/LConn1 -- _CN_183212853_400000_CN_107937167_400000/RConn1
  T_107937167_400000_Delphi_Substation/LConn2 -- _CN_183212853_400000_CN_107937167_400000/RConn2
  _CN_183212853_400000_CN_107937167_400000/RConn3 -- T_107937167_400000_Delphi_Substation/LConn3 -- bus235/LConn1
  T_162871098_400000_Aggeneys_Substation/LConn1 -- _CN_162871098_400000_CN_125769921_400000/LConn1
  T_162871098_400000_Aggeneys_Substation/LConn2 -- _CN_162871098_400000_CN_125769921_400000/LConn2
  _CN_162871098_400000_CN_125769921_400000/LConn3 -- T_162871098_400000_Aggeneys_Substation/LConn3 -- bus236/LConn1
  _CN_162871098_400000_CN_125769921_400000/RConn1 -- T_125769921_400000_Aries_Substation/LConn1 -- _CN_125769921_400000_CN_183402339_400000/LConn1
  _CN_162871098_400000_CN_125769921_400000/RConn2 -- T_125769921_400000_Aries_Substation/LConn2 -- _CN_125769921_400000_CN_183402339_400000/LConn2
  _CN_162871098_400000_CN_125769921_400000/RConn3 -- T_125769921_400000_Aries_Substation/LConn3 -- _CN_125769921_400000_CN_183402339_400000/LConn3 -- bus237/LConn1
  _CN_185171518_400000_CN_185171511_400000/RConn1 -- T_185171518__/LConn1 -- _CN_185171518_400000_CN_75136015_400000/RConn1 -- _CN_185171518_400000_CN_83525879_400000/RConn1
  _CN_185171518_400000_CN_185171511_400000/RConn2 -- T_185171518__/LConn2 -- _CN_185171518_400000_CN_75136015_400000/RConn2 -- _CN_185171518_400000_CN_83525879_400000/RConn2
  _CN_185171518_400000_CN_185171511_400000/RConn3 -- T_185171518__/LConn3 -- _CN_185171518_400000_CN_75136015_400000/RConn3 -- _CN_185171518_400000_CN_83525879_400000/RConn3 -- bus238/LConn1
  _CN_125769921_400000_CN_183402339_400000/RConn1 -- T_183402339_400000_Kronos_Substation/LConn1 -- _CN_183402339_400000_CN_142414070_400000/RConn1
  _CN_125769921_400000_CN_183402339_400000/RConn2 -- T_183402339_400000_Kronos_Substation/LConn2 -- _CN_183402339_400000_CN_142414070_400000/RConn2
  _CN_125769921_400000_CN_183402339_400000/RConn3 -- T_183402339_400000_Kronos_Substation/LConn3 -- _CN_183402339_400000_CN_142414070_400000/RConn3 -- bus239/LConn1
  T_207991752__/LConn1 -- _CN_207991752_400000_CN_176362710_400000/RConn1
  T_207991752__/LConn2 -- _CN_207991752_400000_CN_176362710_400000/RConn2
  _CN_207991752_400000_CN_176362710_400000/RConn3 -- T_207991752__/LConn3 -- bus240/LConn1
  _CN_178882935_400000_CN_75136015_400000/RConn1 -- T_178882935__/LConn1 -- _CN_178882935_400000_CN_87404898_400000/RConn1
  _CN_178882935_400000_CN_75136015_400000/RConn2 -- T_178882935__/LConn2 -- _CN_178882935_400000_CN_87404898_400000/RConn2
  _CN_178882935_400000_CN_75136015_400000/RConn3 -- T_178882935__/LConn3 -- _CN_178882935_400000_CN_87404898_400000/RConn3 -- bus241/LConn1
  T_102682082_400000_Palmiet_Substation/LConn1 -- _CN_102682082_400000_CN_120584910_400000/RConn1
  T_102682082_400000_Palmiet_Substation/LConn2 -- _CN_102682082_400000_CN_120584910_400000/RConn2
  _CN_102682082_400000_CN_120584910_400000/RConn3 -- T_102682082_400000_Palmiet_Substation/LConn3 -- bus242/LConn1
  T_169789536__/LConn1 -- _CN_169789536_400000_CN_121995134_400000/RConn1
  T_169789536__/LConn2 -- _CN_169789536_400000_CN_121995134_400000/RConn2
  _CN_169789536_400000_CN_121995134_400000/RConn3 -- T_169789536__/LConn3 -- bus243/LConn1
  T_209976655__/LConn1 -- _CN_209976655_400000_CN_418832508_275000/RConn1
  T_209976655__/LConn2 -- _CN_209976655_400000_CN_418832508_275000/RConn2
  _CN_209976655_400000_CN_418832508_275000/RConn3 -- T_209976655__/LConn3 -- bus244/LConn1
  _CN_90454383_400000_CN_89637370_400000/RConn1 -- T_89637370_400000_Poseidon_Main_Transmission_Substation/LConn1 -- _CN_142414070_400000_CN_89637370_400000/RConn1
  _CN_90454383_400000_CN_89637370_400000/RConn2 -- T_89637370_400000_Poseidon_Main_Transmission_Substation/LConn2 -- _CN_142414070_400000_CN_89637370_400000/RConn2
  _CN_90454383_400000_CN_89637370_400000/RConn3 -- T_89637370_400000_Poseidon_Main_Transmission_Substation/LConn3 -- _CN_142414070_400000_CN_89637370_400000/RConn3 -- bus245/LConn1
  _CN_107431792_400000_CN_252396496_132000/RConn1 -- T_107431792_400000_Aurora_Substation/LConn1 -- _CN_107431792_400000_CN_193978748_400000/LConn1
  _CN_107431792_400000_CN_252396496_132000/RConn2 -- T_107431792_400000_Aurora_Substation/LConn2 -- _CN_107431792_400000_CN_193978748_400000/LConn2
  _CN_107431792_400000_CN_252396496_132000/RConn3 -- T_107431792_400000_Aurora_Substation/LConn3 -- _CN_107431792_400000_CN_193978748_400000/LConn3 -- bus246/LConn1
  T_193978748_400000_Juno_Substation/LConn1 -- _CN_107431792_400000_CN_193978748_400000/RConn1
  T_193978748_400000_Juno_Substation/LConn2 -- _CN_107431792_400000_CN_193978748_400000/RConn2
  _CN_107431792_400000_CN_193978748_400000/RConn3 -- T_193978748_400000_Juno_Substation/LConn3 -- bus247/LConn1
  _CN_220129604_400000_CN_418832508_275000/RConn1 -- T_220129604_400000_Arnot_Power_Station/LConn1 -- _CN_220129604_400000_CN_185341297_400000/RConn1
  _CN_220129604_400000_CN_418832508_275000/RConn2 -- T_220129604_400000_Arnot_Power_Station/LConn2 -- _CN_220129604_400000_CN_185341297_400000/RConn2
  _CN_220129604_400000_CN_418832508_275000/RConn3 -- T_220129604_400000_Arnot_Power_Station/LConn3 -- _CN_220129604_400000_CN_185341297_400000/RConn3 -- bus248/LConn1
  _CN_92348290_765000_CN_167540668_765000/LConn1 -- T_92348290_400000;275000_Perseus_Substation/LConn1 -- _CN_92348290_765000_CN_193977981_765000/LConn1
  _CN_92348290_765000_CN_167540668_765000/LConn2 -- T_92348290_400000;275000_Perseus_Substation/LConn2 -- _CN_92348290_765000_CN_193977981_765000/LConn2
  _CN_92348290_765000_CN_167540668_765000/LConn3 -- T_92348290_400000;275000_Perseus_Substation/LConn3 -- _CN_92348290_765000_CN_193977981_765000/LConn3 -- bus249/LConn1
  _CN_92348290_765000_CN_167540668_765000/RConn1 -- T_167540668_400000_/LConn1 -- _CN_178968761_765000_CN_167540668_765000/LConn1
  _CN_92348290_765000_CN_167540668_765000/RConn2 -- T_167540668_400000_/LConn2 -- _CN_178968761_765000_CN_167540668_765000/LConn2
  _CN_92348290_765000_CN_167540668_765000/RConn3 -- T_167540668_400000_/LConn3 -- _CN_178968761_765000_CN_167540668_765000/LConn3 -- bus250/LConn1
  _CN_92348290_765000_CN_193977981_765000/RConn1 -- T_193977981__/LConn1 -- _CN_181366662_765000_CN_193977981_765000/LConn1
  _CN_92348290_765000_CN_193977981_765000/RConn2 -- T_193977981__/LConn2 -- _CN_181366662_765000_CN_193977981_765000/LConn2
  _CN_92348290_765000_CN_193977981_765000/RConn3 -- T_193977981__/LConn3 -- _CN_181366662_765000_CN_193977981_765000/LConn3 -- bus251/LConn1
  _CN_181366662_765000_CN_179136373_765000/LConn1 -- T_181366662_400000_Beta_Substation/LConn1 -- _CN_181366662_765000_CN_193977981_765000/RConn1
  _CN_181366662_765000_CN_179136373_765000/LConn2 -- T_181366662_400000_Beta_Substation/LConn2 -- _CN_181366662_765000_CN_193977981_765000/RConn2
  _CN_181366662_765000_CN_179136373_765000/LConn3 -- T_181366662_400000_Beta_Substation/LConn3 -- _CN_181366662_765000_CN_193977981_765000/RConn3 -- bus252/LConn1
  T_179136373__/LConn1 -- _CN_181366662_765000_CN_179136373_765000/RConn1
  T_179136373__/LConn2 -- _CN_181366662_765000_CN_179136373_765000/RConn2
  _CN_181366662_765000_CN_179136373_765000/RConn3 -- T_179136373__/LConn3 -- bus253/LConn1
  T_178968761_765000;400000_/LConn1 -- _CN_178968761_765000_CN_167540668_765000/RConn1
  T_178968761_765000;400000_/LConn2 -- _CN_178968761_765000_CN_167540668_765000/RConn2
  _CN_178968761_765000_CN_167540668_765000/RConn3 -- T_178968761_765000;400000_/LConn3 -- bus254/LConn1
  T_62216709__/RConn1 -- L_62216709/LConn1
  T_62216709__/RConn2 -- L_62216709/LConn2
  L_62216709/LConn3 -- T_62216709__/RConn3 -- bus255/LConn1
  T_402366747__/RConn1 -- L_402366747/LConn1
  T_402366747__/RConn2 -- L_402366747/LConn2
  L_402366747/LConn3 -- T_402366747__/RConn3 -- bus256/LConn1
  T_62208493_132000_Plattekloof_Substation/RConn1 -- L_62208493/LConn1
  T_62208493_132000_Plattekloof_Substation/RConn2 -- L_62208493/LConn2
  L_62208493/LConn3 -- T_62208493_132000_Plattekloof_Substation/RConn3 -- bus257/LConn1
  T_89824175__/RConn1 -- L_89824175/LConn1
  T_89824175__/RConn2 -- L_89824175/LConn2
  L_89824175/LConn3 -- T_89824175__/RConn3 -- bus258/LConn1
  T_189101371__/RConn1 -- L_189101371/LConn1
  T_189101371__/RConn2 -- L_189101371/LConn2
  L_189101371/LConn3 -- T_189101371__/RConn3 -- bus259/LConn1
  T_84198429_132000_/RConn1 -- L_84198429/LConn1
  T_84198429_132000_/RConn2 -- L_84198429/LConn2
  L_84198429/LConn3 -- T_84198429_132000_/RConn3 -- bus260/LConn1
  T_84273857_132000_/RConn1 -- L_84273857/LConn1
  T_84273857_132000_/RConn2 -- L_84273857/LConn2
  L_84273857/LConn3 -- T_84273857_132000_/RConn3 -- bus261/LConn1
  T_84198438__/RConn1 -- L_84198438/LConn1
  T_84198438__/RConn2 -- L_84198438/LConn2
  L_84198438/LConn3 -- T_84198438__/RConn3 -- bus262/LConn1
  T_107673634__/RConn1 -- L_107673634/LConn1
  T_107673634__/RConn2 -- L_107673634/LConn2
  L_107673634/LConn3 -- T_107673634__/RConn3 -- bus263/LConn1
  T_107669638__/RConn1 -- L_107669638/LConn1
  T_107669638__/RConn2 -- L_107669638/LConn2
  L_107669638/LConn3 -- T_107669638__/RConn3 -- bus264/LConn1
  T_84198444_132000_/RConn1 -- L_84198444/LConn1
  T_84198444_132000_/RConn2 -- L_84198444/LConn2
  L_84198444/LConn3 -- T_84198444_132000_/RConn3 -- bus265/LConn1
  T_230496819__/RConn1 -- L_230496819/LConn1
  T_230496819__/RConn2 -- L_230496819/LConn2
  L_230496819/LConn3 -- T_230496819__/RConn3 -- bus266/LConn1
  T_184212847__/RConn1 -- L_184212847/LConn1
  T_184212847__/RConn2 -- L_184212847/LConn2
  L_184212847/LConn3 -- T_184212847__/RConn3 -- bus267/LConn1
  T_84830388__/RConn1 -- L_84830388/LConn1
  T_84830388__/RConn2 -- L_84830388/LConn2
  L_84830388/LConn3 -- T_84830388__/RConn3 -- bus268/LConn1
  T_84830394_132000_/RConn1 -- L_84830394/LConn1
  T_84830394_132000_/RConn2 -- L_84830394/LConn2
  L_84830394/LConn3 -- T_84830394_132000_/RConn3 -- bus269/LConn1
  T_216269407_132000_Belhar_Substation/RConn1 -- L_216269407/LConn1
  T_216269407_132000_Belhar_Substation/RConn2 -- L_216269407/LConn2
  L_216269407/LConn3 -- T_216269407_132000_Belhar_Substation/RConn3 -- bus270/LConn1
  T_118989798_132000_Sarepta_Substation/RConn1 -- L_118989798/LConn1
  T_118989798_132000_Sarepta_Substation/RConn2 -- L_118989798/LConn2
  L_118989798/LConn3 -- T_118989798_132000_Sarepta_Substation/RConn3 -- bus271/LConn1
  T_168366146__/RConn1 -- L_168366146/LConn1
  T_168366146__/RConn2 -- L_168366146/LConn2
  L_168366146/LConn3 -- T_168366146__/RConn3 -- bus272/LConn1
  T_88446823__/RConn1 -- L_88446823/LConn1
  T_88446823__/RConn2 -- L_88446823/LConn2
  L_88446823/LConn3 -- T_88446823__/RConn3 -- bus273/LConn1
  T_107422789_132000_Malmesbury_Substation/RConn1 -- L_107422789/LConn1
  T_107422789_132000_Malmesbury_Substation/RConn2 -- L_107422789/LConn2
  L_107422789/LConn3 -- T_107422789_132000_Malmesbury_Substation/RConn3 -- bus274/LConn1
  T_107431775_132000_Moorreesburg_Substation/RConn1 -- L_107431775/LConn1
  T_107431775_132000_Moorreesburg_Substation/RConn2 -- L_107431775/LConn2
  L_107431775/LConn3 -- T_107431775_132000_Moorreesburg_Substation/RConn3 -- bus275/LConn1
  T_89830761__/RConn1 -- L_89830761/LConn1
  T_89830761__/RConn2 -- L_89830761/LConn2
  L_89830761/LConn3 -- T_89830761__/RConn3 -- bus276/LConn1
  T_184602703__/RConn1 -- L_184602703/LConn1
  T_184602703__/RConn2 -- L_184602703/LConn2
  L_184602703/LConn3 -- T_184602703__/RConn3 -- bus277/LConn1
  T_184646329__/RConn1 -- L_184646329/LConn1
  T_184646329__/RConn2 -- L_184646329/LConn2
  L_184646329/LConn3 -- T_184646329__/RConn3 -- bus278/LConn1
  T_220079546_132000_Firgrove_Substation/RConn1 -- L_220079546/LConn1
  T_220079546_132000_Firgrove_Substation/RConn2 -- L_220079546/LConn2
  L_220079546/LConn3 -- T_220079546_132000_Firgrove_Substation/RConn3 -- bus279/LConn1
  T_204050015__/RConn1 -- L_204050015/LConn1
  T_204050015__/RConn2 -- L_204050015/LConn2
  L_204050015/LConn3 -- T_204050015__/RConn3 -- bus280/LConn1
  T_200223219__/RConn1 -- L_200223219/LConn1
  T_200223219__/RConn2 -- L_200223219/LConn2
  L_200223219/LConn3 -- T_200223219__/RConn3 -- bus281/LConn1
  T_204050024__/RConn1 -- L_204050024/LConn1
  T_204050024__/RConn2 -- L_204050024/LConn2
  L_204050024/LConn3 -- T_204050024__/RConn3 -- bus282/LConn1
  T_183615847__/RConn1 -- L_183615847/LConn1
  T_183615847__/RConn2 -- L_183615847/LConn2
  L_183615847/LConn3 -- T_183615847__/RConn3 -- bus283/LConn1
  T_91979994__/RConn1 -- L_91979994/LConn1
  T_91979994__/RConn2 -- L_91979994/LConn2
  L_91979994/LConn3 -- T_91979994__/RConn3 -- bus284/LConn1
  T_91980007__/RConn1 -- L_91980007/LConn1
  T_91980007__/RConn2 -- L_91980007/LConn2
  L_91980007/LConn3 -- T_91980007__/RConn3 -- bus285/LConn1
  T_213573238__/RConn1 -- L_213573238/LConn1
  T_213573238__/RConn2 -- L_213573238/LConn2
  L_213573238/LConn3 -- T_213573238__/RConn3 -- bus286/LConn1
  T_239878601_132000_/RConn1 -- L_239878601/LConn1
  T_239878601_132000_/RConn2 -- L_239878601/LConn2
  L_239878601/LConn3 -- T_239878601_132000_/RConn3 -- bus287/LConn1
  T_83247270_132000_/RConn1 -- L_83247270/LConn1
  T_83247270_132000_/RConn2 -- L_83247270/LConn2
  L_83247270/LConn3 -- T_83247270_132000_/RConn3 -- bus288/LConn1
  T_337464444_132000_Mtubatuba_Substation/RConn1 -- L_337464444/LConn1
  T_337464444_132000_Mtubatuba_Substation/RConn2 -- L_337464444/LConn2
  L_337464444/LConn3 -- T_337464444_132000_Mtubatuba_Substation/RConn3 -- bus289/LConn1
  T_337464445_132000_Nseleni_Substation/RConn1 -- L_337464445/LConn1
  T_337464445_132000_Nseleni_Substation/RConn2 -- L_337464445/LConn2
  L_337464445/LConn3 -- T_337464445_132000_Nseleni_Substation/RConn3 -- bus290/LConn1
  T_107669635__/RConn1 -- L_107669635/LConn1
  T_107669635__/RConn2 -- L_107669635/LConn2
  L_107669635/LConn3 -- T_107669635__/RConn3 -- bus291/LConn1
  T_107493834_132000;66000_Blouwater_Substation/RConn1 -- L_107493834/LConn1
  T_107493834_132000;66000_Blouwater_Substation/RConn2 -- L_107493834/LConn2
  L_107493834/LConn3 -- T_107493834_132000;66000_Blouwater_Substation/RConn3 -- bus292/LConn1
  T_167590542__/RConn1 -- L_167590542/LConn1
  T_167590542__/RConn2 -- L_167590542/LConn2
  L_167590542/LConn3 -- T_167590542__/RConn3 -- bus293/LConn1
  T_83537732__/RConn1 -- L_83537732/LConn1
  T_83537732__/RConn2 -- L_83537732/LConn2
  L_83537732/LConn3 -- T_83537732__/RConn3 -- bus294/LConn1
  T_84197350_132000_/RConn1 -- L_84197350/LConn1
  T_84197350_132000_/RConn2 -- L_84197350/LConn2
  L_84197350/LConn3 -- T_84197350_132000_/RConn3 -- bus295/LConn1
  T_84360372_132000_/RConn1 -- L_84360372/LConn1
  T_84360372_132000_/RConn2 -- L_84360372/LConn2
  L_84360372/LConn3 -- T_84360372_132000_/RConn3 -- bus296/LConn1
  T_70586039_132000_/RConn1 -- L_70586039/LConn1
  T_70586039_132000_/RConn2 -- L_70586039/LConn2
  L_70586039/LConn3 -- T_70586039_132000_/RConn3 -- bus297/LConn1
  T_84840271__/RConn1 -- L_84840271/LConn1
  T_84840271__/RConn2 -- L_84840271/LConn2
  L_84840271/LConn3 -- T_84840271__/RConn3 -- bus298/LConn1
  T_84273851_132000_/RConn1 -- L_84273851/LConn1
  T_84273851_132000_/RConn2 -- L_84273851/LConn2
  L_84273851/LConn3 -- T_84273851_132000_/RConn3 -- bus299/LConn1
  T_84274096_132000_/RConn1 -- L_84274096/LConn1
  T_84274096_132000_/RConn2 -- L_84274096/LConn2
  L_84274096/LConn3 -- T_84274096_132000_/RConn3 -- bus300/LConn1
  T_84273858_132000_/RConn1 -- L_84273858/LConn1
  T_84273858_132000_/RConn2 -- L_84273858/LConn2
  L_84273858/LConn3 -- T_84273858_132000_/RConn3 -- bus301/LConn1
  T_62219472__/RConn1 -- L_62219472/LConn1
  T_62219472__/RConn2 -- L_62219472/LConn2
  L_62219472/LConn3 -- T_62219472__/RConn3 -- bus302/LConn1
  T_243489615__/RConn1 -- L_243489615/LConn1
  T_243489615__/RConn2 -- L_243489615/LConn2
  L_243489615/LConn3 -- T_243489615__/RConn3 -- bus303/LConn1
  T_91979987__/RConn1 -- L_91979987/LConn1
  T_91979987__/RConn2 -- L_91979987/LConn2
  L_91979987/LConn3 -- T_91979987__/RConn3 -- bus304/LConn1
  T_103754184__/RConn1 -- L_103754184/LConn1
  T_103754184__/RConn2 -- L_103754184/LConn2
  L_103754184/LConn3 -- T_103754184__/RConn3 -- bus305/LConn1
  T_81813288__/RConn1 -- L_81813288/LConn1
  T_81813288__/RConn2 -- L_81813288/LConn2
  L_81813288/LConn3 -- T_81813288__/RConn3 -- bus306/LConn1
  T_171699035__/RConn1 -- L_171699035/LConn1
  T_171699035__/RConn2 -- L_171699035/LConn2
  L_171699035/LConn3 -- T_171699035__/RConn3 -- bus307/LConn1
  T_91979995__/RConn1 -- L_91979995/LConn1
  T_91979995__/RConn2 -- L_91979995/LConn2
  L_91979995/LConn3 -- T_91979995__/RConn3 -- bus308/LConn1
  T_169667549__/RConn1 -- L_169667549/LConn1
  T_169667549__/RConn2 -- L_169667549/LConn2
  L_169667549/LConn3 -- T_169667549__/RConn3 -- bus309/LConn1
  T_217505022__/RConn1 -- L_217505022/LConn1
  T_217505022__/RConn2 -- L_217505022/LConn2
  L_217505022/LConn3 -- T_217505022__/RConn3 -- bus310/LConn1
  T_217505026__/RConn1 -- L_217505026/LConn1
  T_217505026__/RConn2 -- L_217505026/LConn2
  L_217505026/LConn3 -- T_217505026__/RConn3 -- bus311/LConn1
  T_59037450_132000_/RConn1 -- L_59037450/LConn1
  T_59037450_132000_/RConn2 -- L_59037450/LConn2
  L_59037450/LConn3 -- T_59037450_132000_/RConn3 -- bus312/LConn1
  T_262495875__/RConn1 -- L_262495875/LConn1
  T_262495875__/RConn2 -- L_262495875/LConn2
  L_262495875/LConn3 -- T_262495875__/RConn3 -- bus313/LConn1
  T_185153858__/RConn1 -- L_185153858/LConn1
  T_185153858__/RConn2 -- L_185153858/LConn2
  L_185153858/LConn3 -- T_185153858__/RConn3 -- bus314/LConn1
  T_171699034__/RConn1 -- L_171699034/LConn1
  T_171699034__/RConn2 -- L_171699034/LConn2
  L_171699034/LConn3 -- T_171699034__/RConn3 -- bus315/LConn1
  T_83188525__/RConn1 -- L_83188525/LConn1
  T_83188525__/RConn2 -- L_83188525/LConn2
  L_83188525/LConn3 -- T_83188525__/RConn3 -- bus316/LConn1
  T_83244979__/RConn1 -- L_83244979/LConn1
  T_83244979__/RConn2 -- L_83244979/LConn2
  L_83244979/LConn3 -- T_83244979__/RConn3 -- bus317/LConn1
  T_89824178__/RConn1 -- L_89824178/LConn1
  T_89824178__/RConn2 -- L_89824178/LConn2
  L_89824178/LConn3 -- T_89824178__/RConn3 -- bus318/LConn1
  T_62218065__/RConn1 -- L_62218065/LConn1
  T_62218065__/RConn2 -- L_62218065/LConn2
  L_62218065/LConn3 -- T_62218065__/RConn3 -- bus319/LConn1
  T_62218069_132000_Mitchell's_Plain_Substation/RConn1 -- L_62218069/LConn1
  T_62218069_132000_Mitchell's_Plain_Substation/RConn2 -- L_62218069/LConn2
  L_62218069/LConn3 -- T_62218069_132000_Mitchell's_Plain_Substation/RConn3 -- bus320/LConn1
  T_100686191__/RConn1 -- L_100686191/LConn1
  T_100686191__/RConn2 -- L_100686191/LConn2
  L_100686191/LConn3 -- T_100686191__/RConn3 -- bus321/LConn1
  T_100686200__/RConn1 -- L_100686200/LConn1
  T_100686200__/RConn2 -- L_100686200/LConn2
  L_100686200/LConn3 -- T_100686200__/RConn3 -- bus322/LConn1
  T_178069885__/RConn1 -- L_178069885/LConn1
  T_178069885__/RConn2 -- L_178069885/LConn2
  L_178069885/LConn3 -- T_178069885__/RConn3 -- bus323/LConn1
  T_84569471_132000_/RConn1 -- L_84569471/LConn1
  T_84569471_132000_/RConn2 -- L_84569471/LConn2
  L_84569471/LConn3 -- T_84569471_132000_/RConn3 -- bus324/LConn1
  T_84569494__/RConn1 -- L_84569494/LConn1
  T_84569494__/RConn2 -- L_84569494/LConn2
  L_84569494/LConn3 -- T_84569494__/RConn3 -- bus325/LConn1
  T_84569484_132000_/RConn1 -- L_84569484/LConn1
  T_84569484_132000_/RConn2 -- L_84569484/LConn2
  L_84569484/LConn3 -- T_84569484_132000_/RConn3 -- bus326/LConn1
  T_84571572_132000_/RConn1 -- L_84571572/LConn1
  T_84571572_132000_/RConn2 -- L_84571572/LConn2
  L_84571572/LConn3 -- T_84571572_132000_/RConn3 -- bus327/LConn1
  T_84197284_132000_/RConn1 -- L_84197284/LConn1
  T_84197284_132000_/RConn2 -- L_84197284/LConn2
  L_84197284/LConn3 -- T_84197284_132000_/RConn3 -- bus328/LConn1
  T_169667552__/RConn1 -- L_169667552/LConn1
  T_169667552__/RConn2 -- L_169667552/LConn2
  L_169667552/LConn3 -- T_169667552__/RConn3 -- bus329/LConn1
  T_156418717__/RConn1 -- L_156418717/LConn1
  T_156418717__/RConn2 -- L_156418717/LConn2
  L_156418717/LConn3 -- T_156418717__/RConn3 -- bus330/LConn1
  T_178987907__/RConn1 -- L_178987907/LConn1
  T_178987907__/RConn2 -- L_178987907/LConn2
  L_178987907/LConn3 -- T_178987907__/RConn3 -- bus331/LConn1
  T_182262936__/RConn1 -- L_182262936/LConn1
  T_182262936__/RConn2 -- L_182262936/LConn2
  L_182262936/LConn3 -- T_182262936__/RConn3 -- bus332/LConn1
  T_92343043_275000_Boundary_Substation/RConn1 -- L_92343043/LConn1
  T_92343043_275000_Boundary_Substation/RConn2 -- L_92343043/LConn2
  L_92343043/LConn3 -- T_92343043_275000_Boundary_Substation/RConn3 -- bus333/LConn1
  T_217505021__/RConn1 -- L_217505021/LConn1
  T_217505021__/RConn2 -- L_217505021/LConn2
  L_217505021/LConn3 -- T_217505021__/RConn3 -- bus334/LConn1
  T_191269219_275000_/RConn1 -- L_191269219/LConn1
  T_191269219_275000_/RConn2 -- L_191269219/LConn2
  L_191269219/LConn3 -- T_191269219_275000_/RConn3 -- bus335/LConn1
  T_182253896__/RConn1 -- L_182253896/LConn1
  T_182253896__/RConn2 -- L_182253896/LConn2
  L_182253896/LConn3 -- T_182253896__/RConn3 -- bus336/LConn1
  T_184191239_275000_Illovo_Substation/RConn1 -- L_184191239/LConn1
  T_184191239_275000_Illovo_Substation/RConn2 -- L_184191239/LConn2
  L_184191239/LConn3 -- T_184191239_275000_Illovo_Substation/RConn3 -- bus337/LConn1
  T_176259936_275000_Georgedale_Substation/RConn1 -- L_176259936/LConn1
  T_176259936_275000_Georgedale_Substation/RConn2 -- L_176259936/LConn2
  L_176259936/LConn3 -- T_176259936_275000_Georgedale_Substation/RConn3 -- bus338/LConn1
  T_184336448__/RConn1 -- L_184336448/LConn1
  T_184336448__/RConn2 -- L_184336448/LConn2
  L_184336448/LConn3 -- T_184336448__/RConn3 -- bus339/LConn1
  T_215459082_275000_Rigi_Substation/RConn1 -- L_215459082/LConn1
  T_215459082_275000_Rigi_Substation/RConn2 -- L_215459082/LConn2
  L_215459082/LConn3 -- T_215459082_275000_Rigi_Substation/RConn3 -- bus340/LConn1
  T_149126524_275000_/RConn1 -- L_149126524/LConn1
  T_149126524_275000_/RConn2 -- L_149126524/LConn2
  L_149126524/LConn3 -- T_149126524_275000_/RConn3 -- bus341/LConn1
  T_98231341_275000_/RConn1 -- L_98231341/LConn1
  T_98231341_275000_/RConn2 -- L_98231341/LConn2
  L_98231341/LConn3 -- T_98231341_275000_/RConn3 -- bus342/LConn1
  T_183907671_275000;132000_Avon_Substation/RConn1 -- L_183907671/LConn1
  T_183907671_275000;132000_Avon_Substation/RConn2 -- L_183907671/LConn2
  L_183907671/LConn3 -- T_183907671_275000;132000_Avon_Substation/RConn3 -- bus343/LConn1
  T_183907662_275000;132000_Ottawa_Substation/RConn1 -- L_183907662/LConn1
  T_183907662_275000;132000_Ottawa_Substation/RConn2 -- L_183907662/LConn2
  L_183907662/LConn3 -- T_183907662_275000;132000_Ottawa_Substation/RConn3 -- bus344/LConn1
  T_184602696__/RConn1 -- L_184602696/LConn1
  T_184602696__/RConn2 -- L_184602696/LConn2
  L_184602696/LConn3 -- T_184602696__/RConn3 -- bus345/LConn1
  T_32509808__Lepini_Substation/RConn1 -- L_32509808/LConn1
  T_32509808__Lepini_Substation/RConn2 -- L_32509808/LConn2
  L_32509808/LConn3 -- T_32509808__Lepini_Substation/RConn3 -- bus346/LConn1
  T_178950118_275000_Craighall_Substation/RConn1 -- L_178950118/LConn1
  T_178950118_275000_Craighall_Substation/RConn2 -- L_178950118/LConn2
  L_178950118/LConn3 -- T_178950118_275000_Craighall_Substation/RConn3 -- bus347/LConn1
  T_187432497__/RConn1 -- L_187432497/LConn1
  T_187432497__/RConn2 -- L_187432497/LConn2
  L_187432497/LConn3 -- T_187432497__/RConn3 -- bus348/LConn1
  T_136019706__/RConn1 -- L_136019706/LConn1
  T_136019706__/RConn2 -- L_136019706/LConn2
  L_136019706/LConn3 -- T_136019706__/RConn3 -- bus349/LConn1
  T_247956792__/RConn1 -- L_247956792/LConn1
  T_247956792__/RConn2 -- L_247956792/LConn2
  L_247956792/LConn3 -- T_247956792__/RConn3 -- bus350/LConn1
  T_183764510__/RConn1 -- L_183764510/LConn1
  T_183764510__/RConn2 -- L_183764510/LConn2
  L_183764510/LConn3 -- T_183764510__/RConn3 -- bus351/LConn1
  T_363326105__/RConn1 -- L_363326105/LConn1
  T_363326105__/RConn2 -- L_363326105/LConn2
  L_363326105/LConn3 -- T_363326105__/RConn3 -- bus352/LConn1
  T_179856840_275000_Komatipoort_Substation/RConn1 -- L_179856840/LConn1
  T_179856840_275000_Komatipoort_Substation/RConn2 -- L_179856840/LConn2
  L_179856840/LConn3 -- T_179856840_275000_Komatipoort_Substation/RConn3 -- bus353/LConn1
  T_148830396__/RConn1 -- L_148830396/LConn1
  T_148830396__/RConn2 -- L_148830396/LConn2
  L_148830396/LConn3 -- T_148830396__/RConn3 -- bus354/LConn1
  T_84391364_275000_Nevis_Substation/RConn1 -- L_84391364/LConn1
  T_84391364_275000_Nevis_Substation/RConn2 -- L_84391364/LConn2
  L_84391364/LConn3 -- T_84391364_275000_Nevis_Substation/RConn3 -- bus355/LConn1
  T_136695854__/RConn1 -- L_136695854/LConn1
  T_136695854__/RConn2 -- L_136695854/LConn2
  L_136695854/LConn3 -- T_136695854__/RConn3 -- bus356/LConn1
  T_136695855__/RConn1 -- L_136695855/LConn1
  T_136695855__/RConn2 -- L_136695855/LConn2
  L_136695855/LConn3 -- T_136695855__/RConn3 -- bus357/LConn1
  T_184187955_275000_Klaarwater_Substation/RConn1 -- L_184187955/LConn1
  T_184187955_275000_Klaarwater_Substation/RConn2 -- L_184187955/LConn2
  L_184187955/LConn3 -- T_184187955_275000_Klaarwater_Substation/RConn3 -- bus358/LConn1
  T_178240540__/RConn1 -- L_178240540/LConn1
  T_178240540__/RConn2 -- L_178240540/LConn2
  L_178240540/LConn3 -- T_178240540__/RConn3 -- bus359/LConn1
  T_100421919__/RConn1 -- L_100421919/LConn1
  T_100421919__/RConn2 -- L_100421919/LConn2
  L_100421919/LConn3 -- T_100421919__/RConn3 -- bus360/LConn1
  T_200757306__/RConn1 -- L_200757306/LConn1
  T_200757306__/RConn2 -- L_200757306/LConn2
  L_200757306/LConn3 -- T_200757306__/RConn3 -- bus361/LConn1
  T_197060002__/RConn1 -- L_197060002/LConn1
  T_197060002__/RConn2 -- L_197060002/LConn2
  L_197060002/LConn3 -- T_197060002__/RConn3 -- bus362/LConn1
  T_101150274__/RConn1 -- L_101150274/LConn1
  T_101150274__/RConn2 -- L_101150274/LConn2
  L_101150274/LConn3 -- T_101150274__/RConn3 -- bus363/LConn1
  T_138280477__/RConn1 -- L_138280477/LConn1
  T_138280477__/RConn2 -- L_138280477/LConn2
  L_138280477/LConn3 -- T_138280477__/RConn3 -- bus364/LConn1
  T_28088740_275000_Croydon_Substation/RConn1 -- L_28088740/LConn1
  T_28088740_275000_Croydon_Substation/RConn2 -- L_28088740/LConn2
  L_28088740/LConn3 -- T_28088740_275000_Croydon_Substation/RConn3 -- bus365/LConn1
  T_42209860_275000_Jupiter_Substation/RConn1 -- L_42209860/LConn1
  T_42209860_275000_Jupiter_Substation/RConn2 -- L_42209860/LConn2
  L_42209860/LConn3 -- T_42209860_275000_Jupiter_Substation/RConn3 -- bus366/LConn1
  T_178240552__/RConn1 -- L_178240552/LConn1
  T_178240552__/RConn2 -- L_178240552/LConn2
  L_178240552/LConn3 -- T_178240552__/RConn3 -- bus367/LConn1
  T_83945972__/RConn1 -- L_83945972/LConn1
  T_83945972__/RConn2 -- L_83945972/LConn2
  L_83945972/LConn3 -- T_83945972__/RConn3 -- bus368/LConn1
  T_93158442_275000_Marathon_Substation/RConn1 -- L_93158442/LConn1
  T_93158442_275000_Marathon_Substation/RConn2 -- L_93158442/LConn2
  L_93158442/LConn3 -- T_93158442_275000_Marathon_Substation/RConn3 -- bus369/LConn1
  T_178983951__/RConn1 -- L_178983951/LConn1
  T_178983951__/RConn2 -- L_178983951/LConn2
  L_178983951/LConn3 -- T_178983951__/RConn3 -- bus370/LConn1
  T_214437948_275000_Brenner_Substation/RConn1 -- L_214437948/LConn1
  T_214437948_275000_Brenner_Substation/RConn2 -- L_214437948/LConn2
  L_214437948/LConn3 -- T_214437948_275000_Brenner_Substation/RConn3 -- bus371/LConn1
  T_81817181_275000_Eiger_Substation/RConn1 -- L_81817181/LConn1
  T_81817181_275000_Eiger_Substation/RConn2 -- L_81817181/LConn2
  L_81817181/LConn3 -- T_81817181_275000_Eiger_Substation/RConn3 -- bus372/LConn1
  T_189739076_275000_Makalu_Substation/RConn1 -- L_189739076/LConn1
  T_189739076_275000_Makalu_Substation/RConn2 -- L_189739076/LConn2
  L_189739076/LConn3 -- T_189739076_275000_Makalu_Substation/RConn3 -- bus373/LConn1
  T_135726365__/RConn1 -- L_135726365/LConn1
  T_135726365__/RConn2 -- L_135726365/LConn2
  L_135726365/LConn3 -- T_135726365__/RConn3 -- bus374/LConn1
  T_104071861__/RConn1 -- L_104071861/LConn1
  T_104071861__/RConn2 -- L_104071861/LConn2
  L_104071861/LConn3 -- T_104071861__/RConn3 -- bus375/LConn1
  T_185481654__/RConn1 -- L_185481654/LConn1
  T_185481654__/RConn2 -- L_185481654/LConn2
  L_185481654/LConn3 -- T_185481654__/RConn3 -- bus376/LConn1
  T_209979772__/RConn1 -- L_209979772/LConn1
  T_209979772__/RConn2 -- L_209979772/LConn2
  L_209979772/LConn3 -- T_209979772__/RConn3 -- bus377/LConn1
  T_181284056_275000_/RConn1 -- L_181284056/LConn1
  T_181284056_275000_/RConn2 -- L_181284056/LConn2
  L_181284056/LConn3 -- T_181284056_275000_/RConn3 -- bus378/LConn1
  T_83525876__/RConn1 -- L_83525876/LConn1
  T_83525876__/RConn2 -- L_83525876/LConn2
  L_83525876/LConn3 -- T_83525876__/RConn3 -- bus379/LConn1
  T_105811509_275000_Verdun_Substation/RConn1 -- L_105811509/LConn1
  T_105811509_275000_Verdun_Substation/RConn2 -- L_105811509/LConn2
  L_105811509/LConn3 -- T_105811509_275000_Verdun_Substation/RConn3 -- bus380/LConn1
  T_178248302_275000_Kookfontein_Substation/RConn1 -- L_178248302/LConn1
  T_178248302_275000_Kookfontein_Substation/RConn2 -- L_178248302/LConn2
  L_178248302/LConn3 -- T_178248302_275000_Kookfontein_Substation/RConn3 -- bus381/LConn1
  T_178944143_275000_Fordsburg_Substation/RConn1 -- L_178944143/LConn1
  T_178944143_275000_Fordsburg_Substation/RConn2 -- L_178944143/LConn2
  L_178944143/LConn3 -- T_178944143_275000_Fordsburg_Substation/RConn3 -- bus382/LConn1
  T_178252032_275000_Scafell_Substation/RConn1 -- L_178252032/LConn1
  T_178252032_275000_Scafell_Substation/RConn2 -- L_178252032/LConn2
  L_178252032/LConn3 -- T_178252032_275000_Scafell_Substation/RConn3 -- bus383/LConn1
  T_83888980__/RConn1 -- L_83888980/LConn1
  T_83888980__/RConn2 -- L_83888980/LConn2
  L_83888980/LConn3 -- T_83888980__/RConn3 -- bus384/LConn1
  T_82014905_275000_Etna_Substation/RConn1 -- L_82014905/LConn1
  T_82014905_275000_Etna_Substation/RConn2 -- L_82014905/LConn2
  L_82014905/LConn3 -- T_82014905_275000_Etna_Substation/RConn3 -- bus385/LConn1
  T_83950316_275000_Benburg_Substation/RConn1 -- L_83950316/LConn1
  T_83950316_275000_Benburg_Substation/RConn2 -- L_83950316/LConn2
  L_83950316/LConn3 -- T_83950316_275000_Benburg_Substation/RConn3 -- bus386/LConn1
  T_184581460__/RConn1 -- L_184581460/LConn1
  T_184581460__/RConn2 -- L_184581460/LConn2
  L_184581460/LConn3 -- T_184581460__/RConn3 -- bus387/LConn1
  T_185497473__/RConn1 -- L_185497473/LConn1
  T_185497473__/RConn2 -- L_185497473/LConn2
  L_185497473/LConn3 -- T_185497473__/RConn3 -- bus388/LConn1
  T_142414070_400000_Hydra_Substation/RConn1 -- L_142414070/LConn1
  T_142414070_400000_Hydra_Substation/RConn2 -- L_142414070/LConn2
  L_142414070/LConn3 -- T_142414070_400000_Hydra_Substation/RConn3 -- bus389/LConn1
  T_386388564__/RConn1 -- L_386388564/LConn1
  T_386388564__/RConn2 -- L_386388564/LConn2
  L_386388564/LConn3 -- T_386388564__/RConn3 -- bus390/LConn1
  T_184560833__/RConn1 -- L_184560833/LConn1
  T_184560833__/RConn2 -- L_184560833/LConn2
  L_184560833/LConn3 -- T_184560833__/RConn3 -- bus391/LConn1
  T_209365700_400000_/RConn1 -- L_209365700/LConn1
  T_209365700_400000_/RConn2 -- L_209365700/LConn2
  L_209365700/LConn3 -- T_209365700_400000_/RConn3 -- bus392/LConn1
  T_167648085__/RConn1 -- L_167648085/LConn1
  T_167648085__/RConn2 -- L_167648085/LConn2
  L_167648085/LConn3 -- T_167648085__/RConn3 -- bus393/LConn1
  T_104080393__/RConn1 -- L_104080393/LConn1
  T_104080393__/RConn2 -- L_104080393/LConn2
  L_104080393/LConn3 -- T_104080393__/RConn3 -- bus394/LConn1
  T_183759046__/RConn1 -- L_183759046/LConn1
  T_183759046__/RConn2 -- L_183759046/LConn2
  L_183759046/LConn3 -- T_183759046__/RConn3 -- bus395/LConn1
  T_182408147__/RConn1 -- L_182408147/LConn1
  T_182408147__/RConn2 -- L_182408147/LConn2
  L_182408147/LConn3 -- T_182408147__/RConn3 -- bus396/LConn1
  T_98231311_400000_Grootvlei_Substation/RConn1 -- L_98231311/LConn1
  T_98231311_400000_Grootvlei_Substation/RConn2 -- L_98231311/LConn2
  L_98231311/LConn3 -- T_98231311_400000_Grootvlei_Substation/RConn3 -- bus397/LConn1
  T_89173873__/RConn1 -- L_89173873/LConn1
  T_89173873__/RConn2 -- L_89173873/LConn2
  L_89173873/LConn3 -- T_89173873__/RConn3 -- bus398/LConn1
  T_87434264_400000_/RConn1 -- L_87434264/LConn1
  T_87434264_400000_/RConn2 -- L_87434264/LConn2
  L_87434264/LConn3 -- T_87434264_400000_/RConn3 -- bus399/LConn1
  T_184201271__/RConn1 -- L_184201271/LConn1
  T_184201271__/RConn2 -- L_184201271/LConn2
  L_184201271/LConn3 -- T_184201271__/RConn3 -- bus400/LConn1
  T_178240542__/RConn1 -- L_178240542/LConn1
  T_178240542__/RConn2 -- L_178240542/LConn2
  L_178240542/LConn3 -- T_178240542__/RConn3 -- bus401/LConn1
  T_176362710__/RConn1 -- L_176362710/LConn1
  T_176362710__/RConn2 -- L_176362710/LConn2
  L_176362710/LConn3 -- T_176362710__/RConn3 -- bus402/LConn1
  T_105759402__/RConn1 -- L_105759402/LConn1
  T_105759402__/RConn2 -- L_105759402/LConn2
  L_105759402/LConn3 -- T_105759402__/RConn3 -- bus403/LConn1
  T_62193952_400000;132000_Acacia_Park_Substation/RConn1 -- L_62193952/LConn1
  T_62193952_400000;132000_Acacia_Park_Substation/RConn2 -- L_62193952/LConn2
  L_62193952/LConn3 -- T_62193952_400000;132000_Acacia_Park_Substation/RConn3 -- bus404/LConn1
  T_219384657__Omega_Substation/RConn1 -- L_219384657/LConn1
  T_219384657__Omega_Substation/RConn2 -- L_219384657/LConn2
  L_219384657/LConn3 -- T_219384657__Omega_Substation/RConn3 -- bus405/LConn1
  T_121995134_400000_Proteus/RConn1 -- L_121995134/LConn1
  T_121995134_400000_Proteus/RConn2 -- L_121995134/LConn2
  L_121995134/LConn3 -- T_121995134_400000_Proteus/RConn3 -- bus406/LConn1
  T_219596295__/RConn1 -- L_219596295/LConn1
  T_219596295__/RConn2 -- L_219596295/LConn2
  L_219596295/LConn3 -- T_219596295__/RConn3 -- bus407/LConn1
  T_169647963_400000;220000_Grassridge_Substation/RConn1 -- L_169647963/LConn1
  T_169647963_400000;220000_Grassridge_Substation/RConn2 -- L_169647963/LConn2
  L_169647963/LConn3 -- T_169647963_400000;220000_Grassridge_Substation/RConn3 -- bus408/LConn1
  T_90454383_400000;220000_Grassridge_Substation/RConn1 -- L_90454383/LConn1
  T_90454383_400000;220000_Grassridge_Substation/RConn2 -- L_90454383/LConn2
  L_90454383/LConn3 -- T_90454383_400000;220000_Grassridge_Substation/RConn3 -- bus409/LConn1
  T_179140081_400000_/RConn1 -- L_179140081/LConn1
  T_179140081_400000_/RConn2 -- L_179140081/LConn2
  L_179140081/LConn3 -- T_179140081_400000_/RConn3 -- bus410/LConn1
  T_98218556__/RConn1 -- L_98218556/LConn1
  T_98218556__/RConn2 -- L_98218556/LConn2
  L_98218556/LConn3 -- T_98218556__/RConn3 -- bus411/LConn1
  T_238322344__/RConn1 -- L_238322344/LConn1
  T_238322344__/RConn2 -- L_238322344/LConn2
  L_238322344/LConn3 -- T_238322344__/RConn3 -- bus412/LConn1
  T_183757901__Normandie_Substation/RConn1 -- L_183757901/LConn1
  T_183757901__Normandie_Substation/RConn2 -- L_183757901/LConn2
  L_183757901/LConn3 -- T_183757901__Normandie_Substation/RConn3 -- bus413/LConn1
  T_103079596__/RConn1 -- L_103079596/LConn1
  T_103079596__/RConn2 -- L_103079596/LConn2
  L_103079596/LConn3 -- T_103079596__/RConn3 -- bus414/LConn1
  T_170672051__/RConn1 -- L_170672051/LConn1
  T_170672051__/RConn2 -- L_170672051/LConn2
  L_170672051/LConn3 -- T_170672051__/RConn3 -- bus415/LConn1
  T_65600948__/RConn1 -- L_65600948/LConn1
  T_65600948__/RConn2 -- L_65600948/LConn2
  L_65600948/LConn3 -- T_65600948__/RConn3 -- bus416/LConn1
  T_183212853_400000_Neptune_Main_Transmission_Substation/RConn1 -- L_183212853/LConn1
  T_183212853_400000_Neptune_Main_Transmission_Substation/RConn2 -- L_183212853/LConn2
  L_183212853/LConn3 -- T_183212853_400000_Neptune_Main_Transmission_Substation/RConn3 -- bus417/LConn1
  T_107937167_400000_Delphi_Substation/RConn1 -- L_107937167/LConn1
  T_107937167_400000_Delphi_Substation/RConn2 -- L_107937167/LConn2
  L_107937167/LConn3 -- T_107937167_400000_Delphi_Substation/RConn3 -- bus418/LConn1
  T_162871098_400000_Aggeneys_Substation/RConn1 -- L_162871098/LConn1
  T_162871098_400000_Aggeneys_Substation/RConn2 -- L_162871098/LConn2
  L_162871098/LConn3 -- T_162871098_400000_Aggeneys_Substation/RConn3 -- bus419/LConn1
  T_125769921_400000_Aries_Substation/RConn1 -- L_125769921/LConn1
  T_125769921_400000_Aries_Substation/RConn2 -- L_125769921/LConn2
  L_125769921/LConn3 -- T_125769921_400000_Aries_Substation/RConn3 -- bus420/LConn1
  T_185171518__/RConn1 -- L_185171518/LConn1
  T_185171518__/RConn2 -- L_185171518/LConn2
  L_185171518/LConn3 -- T_185171518__/RConn3 -- bus421/LConn1
  T_183402339_400000_Kronos_Substation/RConn1 -- L_183402339/LConn1
  T_183402339_400000_Kronos_Substation/RConn2 -- L_183402339/LConn2
  L_183402339/LConn3 -- T_183402339_400000_Kronos_Substation/RConn3 -- bus422/LConn1
  T_207991752__/RConn1 -- L_207991752/LConn1
  T_207991752__/RConn2 -- L_207991752/LConn2
  L_207991752/LConn3 -- T_207991752__/RConn3 -- bus423/LConn1
  T_178882935__/RConn1 -- L_178882935/LConn1
  T_178882935__/RConn2 -- L_178882935/LConn2
  L_178882935/LConn3 -- T_178882935__/RConn3 -- bus424/LConn1
  T_102682082_400000_Palmiet_Substation/RConn1 -- L_102682082/LConn1
  T_102682082_400000_Palmiet_Substation/RConn2 -- L_102682082/LConn2
  L_102682082/LConn3 -- T_102682082_400000_Palmiet_Substation/RConn3 -- bus425/LConn1
  T_169789536__/RConn1 -- L_169789536/LConn1
  T_169789536__/RConn2 -- L_169789536/LConn2
  L_169789536/LConn3 -- T_169789536__/RConn3 -- bus426/LConn1
  T_209976655__/RConn1 -- L_209976655/LConn1
  T_209976655__/RConn2 -- L_209976655/LConn2
  L_209976655/LConn3 -- T_209976655__/RConn3 -- bus427/LConn1
  T_89637370_400000_Poseidon_Main_Transmission_Substation/RConn1 -- L_89637370/LConn1
  T_89637370_400000_Poseidon_Main_Transmission_Substation/RConn2 -- L_89637370/LConn2
  L_89637370/LConn3 -- T_89637370_400000_Poseidon_Main_Transmission_Substation/RConn3 -- bus428/LConn1
  T_193978748_400000_Juno_Substation/RConn1 -- L_193978748/LConn1
  T_193978748_400000_Juno_Substation/RConn2 -- L_193978748/LConn2
  L_193978748/LConn3 -- T_193978748_400000_Juno_Substation/RConn3 -- bus429/LConn1
  T_193977981__/RConn1 -- L_193977981/LConn1
  T_193977981__/RConn2 -- L_193977981/LConn2
  L_193977981/LConn3 -- T_193977981__/RConn3 -- bus430/LConn1
